simulink model "IEEE123bus_v2019b_Phasor_DPL"  (R2019b)
settings: Solver=VariableStepAuto  StartTime=0.0  StopTime=100  FixedStep=Ts  RelTol=1e-3
InitFcn:
  | a=1; % Loading Factor
  | Ts=0.1;% For Delay Blocks in Voltage Regulator Controls
  | 
  | % Simulation data for the IEEE 123 Node Test Feeder model
  | mi2km = 1.60934;%  miles to km conversion
  | ft2km = 0.0003048; % feet to km conversion
  | ms2F = 1*1e-6/(2*pi*60);% microsiemens to Farads conversion
  | 
  | %% Configuration 1
  | % Series Resitance and Reactance - ohm/mile
  | R_1 = [0.4576 0.1560 0.1535;0.1560 0.4666 0.1580;0.1535 0.1580 0.4615];
  | X_1 = [1.0780 0.5017 0.3849;0.5017 1.0482 0.4236;0.3849 0.4236 1.0651];
  | % charging susceptance - microsiemens/mile
  | B_1 = [5.6765 -1.8319 -0.6982;-1.8319 5.9809 -1.1645;-0.6982 -1.1645 5.3971];
  | 
  | R_1 = R_1/mi2km;
  | L_1 = (X_1/(2*pi*60))/mi2km;
  | C_1 =(B_1*ms2F)/mi2km;
  | 
  | %% Configuration 2 - series reactance - ohm/mile
  | R_2 = [0.4666 0.1580 0.1560;0.1580 0.4615 0.1535;0.1560 0.1535 0.4576];
  | X_2 = [1.0482 0.4236 0.5017;0.4236 1.0651 0.3849;0.5017 0.3849 1.0780];
  | % charging susceptance - microsiemens/mile
  | B_2 = [5.9809 -1.1645 -1.8319;-1.1645 5.3971 -0.6982;-1.8319 -0.6982 5.6765];
  | 
  | R_2 = R_2/mi2km;
  | L_2 = (X_2/(2*pi*60))/mi2km;
  | C_2 =(B_2*ms2F)/mi2km;
  | 
  | %% Configuration 3 - series reactance - ohm/mile
  | R_3 = [0.4615 0.1535 0.1580;0.1535 0.4576 0.1560;0.1580 0.1560 0.4666];
  | X_3 = [1.0651 0.3849 0.4236;0.3849 1.0780 0.5017;0.4236 0.5017 1.0482];
  | % charging susceptance - microsiemens/mile
  | B_3 = [5.3971 -0.6982 -1.1645;-0.6982 5.6765 -1.8319; -1.1645 -1.8319 5.9809];
  | 
  | R_3 = R_3/mi2km;
  | L_3 = (X_3/(2*pi*60))/mi2km;
  | C_3 =(B_3*ms2F)/mi2km;
  | 
  | %% Configuration 4 - series reactance - ohm/mile
  | R_4 = [0.4615 0.1580 0.1535;0.1580 0.4666 0.1560;0.1535 0.1560 0.4576];
  | X_4 = [1.0651 0.4236 0.3849;0.4236 1.0482 0.5017;0.3849 0.5017 1.0780];
  | % charging susceptance - microsiemens/mile
  | B_4 = [5.3971 -1.1645 -0.6982;-1.1645 5.9809 -1.8319;-0.6982 -1.8319 5.6765];
  | 
  | R_4 = R_4/mi2km;
  | L_4 = (X_4/(2*pi*60))/mi2km;
  | C_4 =(B_4*ms2F)/mi2km;
  | 
  | %% Configuration 5 - series reactance - ohm/mile
  | R_5 = [0.4666 0.1560 0.1580;0.1560 0.4576 0.1535;0.1580 0.1535 0.4615];
  | X_5 = [1.0482 0.5017 0.4236;0.5017 1.0780 0.3849;0.4236 0.3849 1.0651];
  | % charging susceptance - microsiemens/mile
  | B_5 = [5.9809 -1.8319 -1.1645;-1.8319 5.6765 -0.6982;-1.1645 -0.6982 5.3971];
  | 
  | R_5 = R_5/mi2km;
  | L_5 = (X_5/(2*pi*60))/mi2km;
  | C_5 =(B_5*ms2F)/mi2km;
  | 
  | %% Configuration 6 - series reactance - ohm/mile
  | R_6 = [0.4576 0.1535 0.1560;0.1535 0.4615 0.1580;0.1560 0.1580 0.4666];
  | X_6 = [1.0780 0.3849 0.5017;0.3849 1.0651 0.4236;0.5017 0.4236 1.0482];
  | % charging susceptance - microsiemens/mile
  | B_6 = [5.6765 -0.6982 -1.8319;-0.6982 5.3971 -1.1645;-1.8319 -1.1645 5.9809];
  | 
  | R_6 = R_6/mi2km;
  | L_6 = (X_6/(2*pi*60))/mi2km;
  | C_6 =(B_6*ms2F)/mi2km;
  | 
  | %% Configuration 7 - series reactance - ohm/mile
  | R_7 = [0.4576 0.0000 0.1535;0.0000 0.0000 0.0000;0.1535 0.0000 0.4615];
  | X_7 = [1.0780 0.0000 0.3849;0.0000 0.0000 0.0000;0.3849 0.0000 1.0651];
  | % charging susceptance - microsiemens/mile
  | B_7 = [5.1154 0.0000 -1.0549;0.0000 0.0000 0.0000;-1.0549 0.0000 5.1704];
  | 
  | R_7 = R_7/mi2km;
  | L_7 = (X_7/(2*pi*60))/mi2km;
  | C_7 =(B_7*ms2F)/mi2km;
  | 
  | %% Configuration 8 - series reactance - ohm/mile
  | R_8 = [0.4576 0.1535 0.0000;0.1535 0.4615 0.0000;0.0000 0.0000 0.0000];
  | X_8 = [1.0780 0.3849 0.0000;0.3849 1.0651 0.0000;0.0000 0.0000 0.0000];
  | % charging susceptance - microsiemens/mile
  | B_8 = [5.1154 -1.0549 0.0000;-1.0549 5.1704 0.0000;0.0000 0.0000 0.0000];
  | 
  | R_8 = R_8/mi2km;
  | L_8 = (X_8/(2*pi*60))/mi2km;
  | C_8 =(B_8*ms2F)/mi2km;
  | 
  | %% Configuration 9 - series reactance - ohm/mile
  | R_9 = [1.3292 0 0;0 0 0;0 0 0];
  | X_9 = [1.3475 0 0;0 0 0;0 0 0];
  | % charging susceptance - microsiemens/mile
  | B_9 = [4.5193 0 0;0 0 0;0 0 0];
  | 
  | R_9 = R_9/mi2km;
  | L_9 = (X_9/(2*pi*60))/mi2km;
  | C_9 =(B_9*ms2F)/mi2km;
  | 
  | %% Configuration 10- series reactance - ohm/mile
  | R_10 = [0 0 0;0 1.3292 0;0 0 0];
  | X_10 = [0 0 0;0 1.3475 0;0 0 0];
  | % charging susceptance - microsiemens/mile
  | B_10 = [0 0 0;0 4.5193 0;0 0 0];
  | 
  | R_10 = R_10/mi2km;
  | L_10 = (X_10/(2*pi*60))/mi2km;
  | C_10 =(B_10*ms2F)/mi2km;
  | 
  | %% Configuration 11 - series reactance - ohm/mile
  | R_11 = [0 0 0;0 0 0;0 0 1.3292];
  | X_11 = [0 0 0;0 0 0;0 0 1.3475];
  | % charging susceptance - microsiemens/mile
  | B_11 = [0 0 0;0 0 0;0 0 4.5193];
  | 
  | R_11 = R_11/mi2km;
  | L_11 = (X_11/(2*pi*60))/mi2km;
  | C_11 =(B_11*ms2F)/mi2km;
  | 
  | %% Configuration 12 - series reactance - ohm/mile
  | R_12 = [1.5209 0.5198 0.4924;0.5198 1.5329 0.5198;0.4924 0.5198 1.5209];
  | X_12 = [0.7521 0.2775 0.2157;0.2775 0.7162 0.2775;0.2157 0.2775 0.7521];
  | % charging susceptance - microsiemens/mile
  | B_12 = [67.2242 0.0000 0.0000;0.0000 67.2242 0.0000;0.0000 0.0000 67.2242];
  | 
  | R_12 = R_12/mi2km;
  | L_12 = (X_12/(2*pi*60))/mi2km;
  | C_12 =(B_12*ms2F)/mi2km;
undefined symbols (not defined in the file or in its folder): D1, Delta, find_system, j
libraries: powerlib x686, powerlib_meascontrol x31
(part 1 of 7)
settings Model: ARTEMISmethode_block_infos=$$__separator__$$pi123variableloadwith3PV/ARTEMIS Guide$$__separator__$$  Creator=Arun  LastModifiedBy=USARSUR
settings DataIOCC: ReturnWorkspaceOutputs=off
settings DebuggingCC: UnconnectedInputMsg=none  UnconnectedOutputMsg=none  UnconnectedLineMsg=none  ArithmeticOperatorsInVariantConditions=warning
settings SFSimCC: SimUseLocalCustomCode=off  CustomCodeUndefinedFunction=UseInterfaceOnly
settings RTWCC: RTWUseLocalCustomCode=off
settings CodeAppCC: StateflowObjectComments=on
settings SimscapeCC: SimscapeNormalizeSystem=off

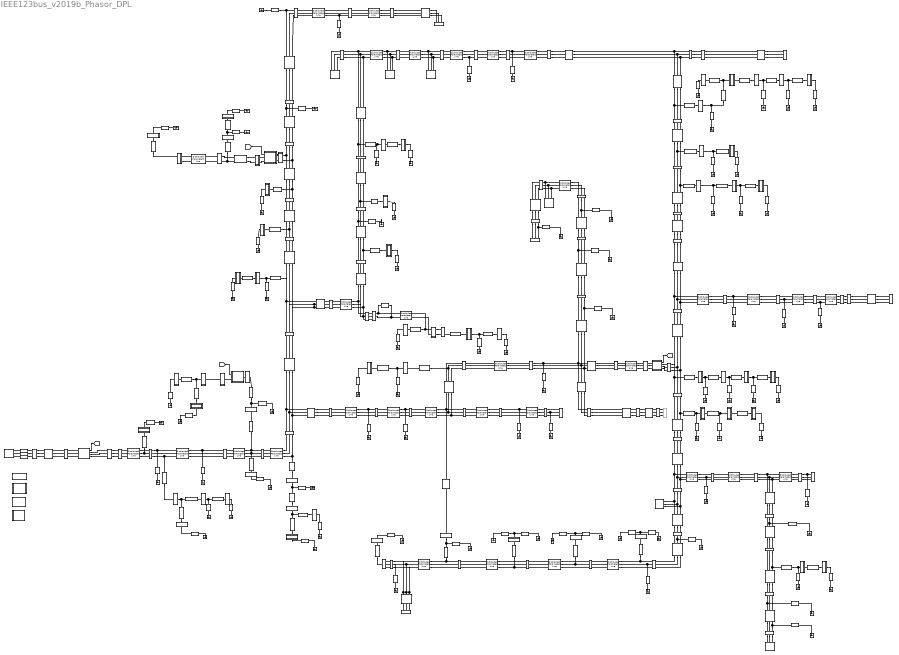
== system IEEE123bus_v2019b_Phasor_DPL ==
  note: Please consider citing following papers if the model was useful for your research
      |
      | A. Suresh, R. Bisht and S. Kamalasadan, "A Coordinated Control Architecture With Inverter-Based Resources and Legacy
      | Controllers of Power Distribution System for Voltage Profile Balance," in IEEE Transactions on Industry Applications, vol. 58,
      | no. 5, pp. 6701-6712, Sept.-Oct. 2022, doi: 10.1109/TIA.2022.3183030.
      |
      | A. Suresh, R. Bisht and S. Kamalasadan, "ADMM Based LQR for Voltage Regulation Using Distributed Energy Resources,"
      | 2020 IEEE International Conference on Power Electronics, Drives and Energy Systems (PEDES), 2020, pp. 1-6,
      | doi: 10.1109/PEDES49360.2020.9379625.
  note: Model Created by
      | Arun Suresh, Dr. Sukumar Kamalasadan,
      | University of North Carolina, Charlotte
  1 : powerlib/Measurements/Three-Phase V-I Measurement  VoltageMeasurement=phase-to-ground  SetLabelV=on  LabelV=V1  Vpu=off  VpuLL=off  CurrentMeasurement=no  SetLabelI=on  LabelI=I800  Ipu=off  Pbase=100e6  Vbase=24900  OutputType=Complex  PhasorSimulation=on  PSBequivalent=0
      settings: SourceProductName=Simscape Electrical
  1 Y PQ : powerlib/Elements/Series RLC Load  LConnTagsString=a  RConnTagsString=__new0  NominalVoltage=1.0*2401.78  NominalFrequency=60  ActivePower=40e3*a  InductivePower=20e3*a  CapacitivePower=0  Setx0=off  InitialVoltage=0  SetiL0=off  InitialCurrent=0  Measurements=None  LoadType=constant PQ
      settings: SourceProductName=Simscape Electrical
  1-2 10 : powerlib/Elements/Distributed Parameters Line  Phases=1  Frequency=60  Resistance=R_10(2,2)  Inductance=L_10(2,2)  Capacitance=C_10(2,2)  Length=175*ft2km  x1=[3380.56541461318;376.991118430775;-2.09963214230387]  x2=[3379.78750747913;376.991118430775;-2.09971060156131]  x3=[8.05427248749283;376.991118430775;0.227346207910768]  x4=[18.8407875620116;376.991118430775;-2.41591493087722]  x5=2.16957196133287e-07  V1=[2.049e+04;377;-2.115]  V2=[2.048e+04;377;-2.115]  I1=[33.62;377;-2.106]  I2=[35.2;377;-2.126]  nHarmo=1  Measurements=None
      settings: SourceProductName=Simscape Electrical
  1-3 11 : powerlib/Elements/Distributed Parameters Line  Phases=1  Frequency=60  Resistance=R_11(3,3)  Inductance=L_11(3,3)  Capacitance=C_11(3,3)  Length=250*ft2km  x1=[3361.50737999427;376.991118430775;2.08819907599433]  x2=[3355.99570274487;376.991118430775;2.08764080595054]  x3=[59.5194469552761;376.991118430775;-1.56433681880081]  x4=[70.5082076019166;376.991118430775;1.66262028833774]  x5=3.09938851618982e-07  V1=[2.049e+04;377;-2.115]  V2=[2.048e+04;377;-2.115]  I1=[33.62;377;-2.106]  I2=[35.2;377;-2.126]  nHarmo=1  Measurements=None
      settings: SourceProductName=Simscape Electrical
  1-7 1 : powerlib/Elements/Distributed Parameters Line  Phases=3  Frequency=60  Resistance=R_1  Inductance=L_1  Capacitance=C_1  Length=300*ft2km  x1=[418.369379874653 4119.59472126334 4115.60124511401;376.991118430775 376.991118430775 376.991118430775;1.71644980792441 -2.40630365835405 2.30078484563816]  x2=[407.597893112689 4096.26742166794 4094.04240143975;376.991118430775 376.991118430775 376.991118430775;1.73955161673438 -2.41014446431971 2.29348797562817]  x3=[123.925310729622 768.405747771136 838.862973764322;376.991118430775 376.991118430775 376.991118430775;2.95122481621433 0.252448117024993 -1.05952038647415]  x4=[123.559999451766 795.721759153579 862.519058134177;376.991118430775 376.991118430775 376.991118430775;-0.182106883383004 -2.87131680733943 2.08805814509585]  x5=3.76244991844366e-07  V1=ones(3,3)  V2=ones(3,3)  I1=ones(3,3)  I2=ones(3,3)  nHarmo=1  Measurements=None
      settings: SourceProductName=Simscape Electrical
  10 : Subsystem
  10 Y I : powerlib/Elements/Series RLC Load  LConnTagsString=a  RConnTagsString=__new0  NominalVoltage=1.0*2401.78  NominalFrequency=60  ActivePower=20e3*a  InductivePower=10e3*a  CapacitivePower=0  Setx0=off  InitialVoltage=0  SetiL0=off  InitialCurrent=0  Measurements=None  LoadType=constant I
      settings: SourceProductName=Simscape Electrical
  100 : powerlib/Measurements/Three-Phase V-I Measurement  VoltageMeasurement=phase-to-ground  SetLabelV=on  LabelV=V100  Vpu=off  VpuLL=off  CurrentMeasurement=no  SetLabelI=on  LabelI=I65  Ipu=off  Pbase=100e6  Vbase=24900  OutputType=Complex  PhasorSimulation=on  PSBequivalent=0
      settings: SourceProductName=Simscape Electrical
  100 Y Z : powerlib/Elements/Series RLC Load  LConnTagsString=a  RConnTagsString=__new0  NominalVoltage=1.0*2401.78  NominalFrequency=60  ActivePower=40e3*a  InductivePower=20e3*a  CapacitivePower=0  Setx0=off  InitialVoltage=0  SetiL0=off  InitialCurrent=0  Measurements=None  LoadType=constant Z
      settings: SourceProductName=Simscape Electrical
  100-450 3 : powerlib/Elements/Distributed Parameters Line  Phases=3  Frequency=60  Resistance=R_3  Inductance=L_3  Capacitance=C_3  Length=800*ft2km  x1=[406.131749441997 3939.12031039649 4017.5206124443;376.991118430775 376.991118430775 376.991118430775;-0.637933141409398 0.171201528668262 1.73700521240345]  x2=[406.131778494139 3939.12050268383 4017.52081027597;376.991118430775 376.991118430775 376.991118430775;-0.637933170107235 0.171201507341509 1.73700518522562]  x3=[0.533763849649707 11.60984734928 14.9950488986919;376.991118430775 376.991118430775 376.991118430775;-0.638311398489514 0.170889060671563 1.73669137648016]  x4=[0.533763849639262 11.6098473492939 14.9950488987535;376.991118430775 376.991118430775 376.991118430775;-0.637933170089052 0.171201507340757 1.73700518522527]  x5=1.00331997825164e-06  V1=ones(3,3)  V2=ones(3,3)  I1=ones(3,3)  I2=ones(3,3)  nHarmo=1  Measurements=None
      settings: SourceProductName=Simscape Electrical
  101 : powerlib/Measurements/Three-Phase V-I Measurement  VoltageMeasurement=phase-to-ground  SetLabelV=on  LabelV=V101  Vpu=off  VpuLL=off  CurrentMeasurement=no  SetLabelI=on  LabelI=I65  Ipu=off  Pbase=100e6  Vbase=24900  OutputType=Complex  PhasorSimulation=on  PSBequivalent=0
      settings: SourceProductName=Simscape Electrical
  101-102 11 : powerlib/Elements/Distributed Parameters Line  Phases=1  Frequency=60  Resistance=R_11(3,3)  Inductance=L_11(3,3)  Capacitance=C_11(3,3)  Length=225*ft2km  x1=[3251.35849286821;376.991118430775;2.0524184497167]  x2=[3246.56346361664;376.991118430775;2.05191677401351]  x3=[57.5262989800154;376.991118430775;-1.60039970533835]  x4=[68.1545739922667;376.991118430775;1.62666785892524]  x5=2.78944966457084e-07  V1=[2.049e+04;377;-2.115]  V2=[2.048e+04;377;-2.115]  I1=[33.62;377;-2.106]  I2=[35.2;377;-2.126]  nHarmo=1  Measurements=None
      settings: SourceProductName=Simscape Electrical
  101-105 3 : powerlib/Elements/Distributed Parameters Line  Phases=3  Frequency=60  Resistance=R_3  Inductance=L_3  Capacitance=C_3  Length=275*ft2km  x1=[403.657094793231 3937.42755462039 4018.23187990053;376.991118430775 376.991118430775 376.991118430775;-0.650924692497019 0.171464273667595 1.73744251449841]  x2=[403.635418531243 3934.47089431162 4016.39907349208;376.991118430775 376.991118430775 376.991118430775;-0.655781561403268 0.170968215664939 1.73704867653885]  x3=[17.9003688107967 79.6160512452646 59.5124978469701;376.991118430775 376.991118430775 376.991118430775;2.86937115405689 2.65811987542283 -1.846283722212]  x4=[18.8894010898735 99.0347590423608 87.5672430146078;376.991118430775 376.991118430775 376.991118430775;-0.293121067652145 -0.340334133509769 1.44230191886661]  x5=3.44891242524002e-07  V1=ones(3,3)  V2=ones(3,3)  I1=ones(3,3)  I2=ones(3,3)  nHarmo=1  Measurements=None
      settings: SourceProductName=Simscape Electrical
  102 : Subsystem
  102 Y Z : powerlib/Elements/Series RLC Load  LConnTagsString=a  RConnTagsString=__new0  NominalVoltage=1.0*2401.78  NominalFrequency=60  ActivePower=20e3*a  InductivePower=10e3*a  CapacitivePower=0  Setx0=off  InitialVoltage=0  SetiL0=off  InitialCurrent=0  Measurements=None  LoadType=constant Z
      settings: SourceProductName=Simscape Electrical
  102-103 11 : powerlib/Elements/Distributed Parameters Line  Phases=1  Frequency=60  Resistance=R_11(3,3)  Inductance=L_11(3,3)  Capacitance=C_11(3,3)  Length=325*ft2km  x1=[3246.56346361664;376.991118430775;2.05187003633578]  x2=[3241.0261246808;376.991118430775;2.05128908924918]  x3=[44.9655499069155;376.991118430775;-1.61347437800645]  x4=[55.5730572774;376.991118430775;1.63516683558841]  x5=4.02920507104677e-07  V1=[2.049e+04;377;-2.115]  V2=[2.048e+04;377;-2.115]  I1=[33.62;377;-2.106]  I2=[35.2;377;-2.126]  nHarmo=1  Measurements=None
      settings: SourceProductName=Simscape Electrical
  103 : Subsystem
  103 Y PQ : powerlib/Elements/Series RLC Load  LConnTagsString=a  RConnTagsString=__new0  NominalVoltage=1.0*2401.78  NominalFrequency=60  ActivePower=40e3*a  InductivePower=20e3*a  CapacitivePower=0  Setx0=off  InitialVoltage=0  SetiL0=off  InitialCurrent=0  Measurements=None  LoadType=constant PQ
      settings: SourceProductName=Simscape Electrical
  103-104 11 : powerlib/Elements/Distributed Parameters Line  Phases=1  Frequency=60  Resistance=R_11(3,3)  Inductance=L_11(3,3)  Capacitance=C_11(3,3)  Length=700*ft2km  x1=[3241.0261246808;376.991118430775;2.05111382295771]  x2=[3235.06887030603;376.991118430775;2.05048713201662]  x3=[19.9470002767371;376.991118430775;-1.68827039446278]  x4=[30.4892896750951;376.991118430775;1.67382868946066]  x5=8.6782878453315e-07  V1=[2.049e+04;377;-2.115]  V2=[2.048e+04;377;-2.115]  I1=[33.62;377;-2.106]  I2=[35.2;377;-2.126]  nHarmo=1  Measurements=None
      settings: SourceProductName=Simscape Electrical
  104 : Subsystem
  104 Y PQ : powerlib/Elements/Series RLC Load  LConnTagsString=a  RConnTagsString=__new0  NominalVoltage=1.0*2401.78  NominalFrequency=60  ActivePower=40e3*a  InductivePower=20e3*a  CapacitivePower=0  Setx0=off  InitialVoltage=0  SetiL0=off  InitialCurrent=0  Measurements=None  LoadType=constant PQ
      settings: SourceProductName=Simscape Electrical
  105 : powerlib/Measurements/Three-Phase V-I Measurement  VoltageMeasurement=phase-to-ground  SetLabelV=on  LabelV=V105  Vpu=off  VpuLL=off  CurrentMeasurement=no  SetLabelI=on  LabelI=I65  Ipu=off  Pbase=100e6  Vbase=24900  OutputType=Complex  PhasorSimulation=on  PSBequivalent=0
      settings: SourceProductName=Simscape Electrical
  105-106 10 : powerlib/Elements/Distributed Parameters Line  Phases=1  Frequency=60  Resistance=R_10(2,2)  Inductance=L_10(2,2)  Capacitance=C_10(2,2)  Length=225*ft2km  x1=[3304.98190011473;376.991118430775;-2.13405919078126]  x2=[3301.07685262134;376.991118430775;-2.13446171946558]  x3=[45.8104144500859;376.991118430775;0.484075429353889]  x4=[56.6127579803776;376.991118430775;-2.55054593205608]  x5=2.78944966457084e-07  V1=[2.049e+04;377;-2.115]  V2=[2.048e+04;377;-2.115]  I1=[33.62;377;-2.106]  I2=[35.2;377;-2.126]  nHarmo=1  Measurements=None
      settings: SourceProductName=Simscape Electrical
  105-108 3 : powerlib/Elements/Distributed Parameters Line  Phases=3  Frequency=60  Resistance=R_3  Inductance=L_3  Capacitance=C_3  Length=325*ft2km  x1=[403.635418531243 3934.47089431162 4016.39907349208;376.991118430775 376.991118430775 376.991118430775;-0.655805201573315 0.1709486870816 1.7370290626429]  x2=[402.074723888673 3931.7722646479 4016.56807334287;376.991118430775 376.991118430775 376.991118430775;-0.671182237047441 0.170609231399958 1.73692119301889]  x3=[50.1878882304407 55.6962408839422 11.7513473466765;376.991118430775 376.991118430775 376.991118430775;2.61416246353745 2.47843227593797 0.843207511127157]  x4=[51.2372486550466 73.3161862808586 24.4058651044384;376.991118430775 376.991118430775 376.991118430775;-0.530234910581878 -0.426773816811748 2.12160754968628]  x5=4.0759874116473e-07  V1=ones(3,3)  V2=ones(3,3)  I1=ones(3,3)  I2=ones(3,3)  nHarmo=1  Measurements=None
      settings: SourceProductName=Simscape Electrical
  106 : Subsystem
  106 Y PQ : powerlib/Elements/Series RLC Load  LConnTagsString=a  RConnTagsString=__new0  NominalVoltage=1.0*2401.78  NominalFrequency=60  ActivePower=40e3*a  InductivePower=20e3*a  CapacitivePower=0  Setx0=off  InitialVoltage=0  SetiL0=off  InitialCurrent=0  Measurements=None  LoadType=constant PQ
      settings: SourceProductName=Simscape Electrical
  106-107 10 : powerlib/Elements/Distributed Parameters Line  Phases=1  Frequency=60  Resistance=R_10(2,2)  Inductance=L_10(2,2)  Capacitance=C_10(2,2)  Length=575*ft2km  x1=[3301.07685262134;376.991118430775;-2.13462530133762]  x2=[3296.09115865668;376.991118430775;-2.13514024446439]  x3=[20.3252283129498;376.991118430775;0.40935318589622]  x4=[31.0653774222284;376.991118430775;-2.51179765756046]  x5=7.12859358723659e-07  V1=[2.049e+04;377;-2.115]  V2=[2.048e+04;377;-2.115]  I1=[33.62;377;-2.106]  I2=[35.2;377;-2.126]  nHarmo=1  Measurements=None
      settings: SourceProductName=Simscape Electrical
  107 : Subsystem
  107 Y PQ : powerlib/Elements/Series RLC Load  LConnTagsString=a  RConnTagsString=__new0  NominalVoltage=1.0*2401.78  NominalFrequency=60  ActivePower=40e3*a  InductivePower=20e3*a  CapacitivePower=0  Setx0=off  InitialVoltage=0  SetiL0=off  InitialCurrent=0  Measurements=None  LoadType=constant PQ
      settings: SourceProductName=Simscape Electrical
  108 : powerlib/Measurements/Three-Phase V-I Measurement  VoltageMeasurement=phase-to-ground  SetLabelV=on  LabelV=V108  Vpu=off  VpuLL=off  CurrentMeasurement=no  SetLabelI=on  LabelI=I65  Ipu=off  Pbase=100e6  Vbase=24900  OutputType=Complex  PhasorSimulation=on  PSBequivalent=0
      settings: SourceProductName=Simscape Electrical
  108-109 9 : powerlib/Elements/Distributed Parameters Line  Phases=1  Frequency=60  Resistance=R_9(1,1)  Inductance=L_9(1,1)  Capacitance=C_9(1,1)  Length=450*ft2km  x1=[3181.15673359339;376.991118430775;-0.0628869901083998]  x2=[3168.06194978621;376.991118430775;-0.0642859616608475]  x3=[80.5463139182893;376.991118430775;2.58026488742804]  x4=[90.9315802089911;376.991118430775;-0.500259322316593]  x5=5.57889932914168e-07  V1=[2.049e+04;377;-2.115]  V2=[2.048e+04;377;-2.115]  I1=[33.62;377;-2.106]  I2=[35.2;377;-2.126]  nHarmo=1  Measurements=None
      settings: SourceProductName=Simscape Electrical
  108-300 3 : powerlib/Elements/Distributed Parameters Line  Phases=3  Frequency=60  Resistance=R_3  Inductance=L_3  Capacitance=C_3  Length=1000*ft2km  x1=[402.074723888673 3931.7722646479 4016.56807334287;376.991118430775 376.991118430775 376.991118430775;-0.671501379343069 0.170345595524886 1.73665640542353]  x2=[402.074761358754 3931.77255721669 4016.56837602683;376.991118430775 376.991118430775 376.991118430775;-0.671501420907049 0.170345564472289 1.73665636432255]  x3=[0.528412808323245 11.5879303032605 14.9910215576854;376.991118430775 376.991118430775 376.991118430775;-0.671937963049553 0.169961143904011 1.73626866977983]  x4=[0.528420850969568 11.5878577029287 14.9909927851014;376.991118430775 376.991118430775 376.991118430775;-0.671537666068559 0.170339428949189 1.73665180118272]  x5=1.25414997281455e-06  V1=ones(3,3)  V2=ones(3,3)  I1=ones(3,3)  I2=ones(3,3)  nHarmo=1  Measurements=None
      settings: SourceProductName=Simscape Electrical
  109 : Subsystem
  109 Y PQ : powerlib/Elements/Series RLC Load  LConnTagsString=a  RConnTagsString=__new0  NominalVoltage=1.0*2401.78  NominalFrequency=60  ActivePower=40e3*a  InductivePower=20e3*a  CapacitivePower=0  Setx0=off  InitialVoltage=0  SetiL0=off  InitialCurrent=0  Measurements=None  LoadType=constant PQ
      settings: SourceProductName=Simscape Electrical
  109-110 9 : powerlib/Elements/Distributed Parameters Line  Phases=1  Frequency=60  Resistance=R_9(1,1)  Inductance=L_9(1,1)  Capacitance=C_9(1,1)  Length=300*ft2km  x1=[3168.06194978621;376.991118430775;-0.0642158551442573]  x2=[3161.83483122911;376.991118430775;-0.064884594025442]  x3=[56.0271358889941;376.991118430775;2.56601096641357]  x4=[66.3801617084479;376.991118430775;-0.490087419533799]  x5=3.71926621942778e-07  V1=[2.049e+04;377;-2.115]  V2=[2.048e+04;377;-2.115]  I1=[33.62;377;-2.106]  I2=[35.2;377;-2.126]  nHarmo=1  Measurements=None
      settings: SourceProductName=Simscape Electrical
  11 : Subsystem
  11 Y Z : powerlib/Elements/Series RLC Load  LConnTagsString=a  RConnTagsString=__new0  NominalVoltage=1.0*2401.78  NominalFrequency=60  ActivePower=40e3*a  InductivePower=20e3*a  CapacitivePower=0  Setx0=off  InitialVoltage=0  SetiL0=off  InitialCurrent=0  Measurements=None  LoadType=constant Z
      settings: SourceProductName=Simscape Electrical
  110 : Subsystem
  110-111 9 : powerlib/Elements/Distributed Parameters Line  Phases=1  Frequency=60  Resistance=R_9(1,1)  Inductance=L_9(1,1)  Capacitance=C_9(1,1)  Length=575*ft2km  x1=[3161.83483122911;376.991118430775;-0.0650131226391907]  x2=[3159.44549174791;376.991118430775;-0.0652708065834279]  x3=[7.52655039714254;376.991118430775;2.26152167646501]  x4=[17.6106029911177;376.991118430775;-0.381479851658474]  x5=7.12859358723659e-07  V1=[2.049e+04;377;-2.115]  V2=[2.048e+04;377;-2.115]  I1=[33.62;377;-2.106]  I2=[35.2;377;-2.126]  nHarmo=1  Measurements=None
      settings: SourceProductName=Simscape Electrical
  110-112 9 : powerlib/Elements/Distributed Parameters Line  Phases=1  Frequency=60  Resistance=R_9(1,1)  Inductance=L_9(1,1)  Capacitance=C_9(1,1)  Length=125*ft2km  x1=[3161.83483122911;376.991118430775;-0.0648028030894201]  x2=[3159.75997373429;376.991118430775;-0.0650261502258887]  x3=[43.8089246818886;376.991118430775;2.55317269137536]  x4=[54.1453656807879;376.991118430775;-0.481335615539711]  x5=1.54969425809491e-07  V1=[2.049e+04;377;-2.115]  V2=[2.048e+04;377;-2.115]  I1=[33.62;377;-2.106]  I2=[35.2;377;-2.126]  nHarmo=1  Measurements=None
      settings: SourceProductName=Simscape Electrical
  111 : Subsystem
  111 Y PQ : powerlib/Elements/Series RLC Load  LConnTagsString=a  RConnTagsString=__new0  NominalVoltage=1.0*2401.78  NominalFrequency=60  ActivePower=20e3*a  InductivePower=10e3*a  CapacitivePower=0  Setx0=off  InitialVoltage=0  SetiL0=off  InitialCurrent=0  Measurements=None  LoadType=constant PQ
      settings: SourceProductName=Simscape Electrical
  112 : Subsystem
  112 Y I : powerlib/Elements/Series RLC Load  LConnTagsString=a  RConnTagsString=__new0  NominalVoltage=1.0*2401.78  NominalFrequency=60  ActivePower=20e3*a  InductivePower=10e3*a  CapacitivePower=0  Setx0=off  InitialVoltage=0  SetiL0=off  InitialCurrent=0  Measurements=None  LoadType=constant I
      settings: SourceProductName=Simscape Electrical
  112-113 9 : powerlib/Elements/Distributed Parameters Line  Phases=1  Frequency=60  Resistance=R_9(1,1)  Inductance=L_9(1,1)  Capacitance=C_9(1,1)  Length=525*ft2km  x1=[3159.75997373429;376.991118430775;-0.0652131009367958]  x2=[3153.22836502941;376.991118430775;-0.0659177727875796]  x3=[31.5914511772632;376.991118430775;2.52992679657941]  x4=[41.9022702912703;376.991118430775;-0.467929617642989]  x5=6.50871588399862e-07  V1=[2.049e+04;377;-2.115]  V2=[2.048e+04;377;-2.115]  I1=[33.62;377;-2.106]  I2=[35.2;377;-2.126]  nHarmo=1  Measurements=None
      settings: SourceProductName=Simscape Electrical
  113 : Subsystem
  113 Y Z : powerlib/Elements/Series RLC Load  LConnTagsString=a  RConnTagsString=__new0  NominalVoltage=1.0*2401.78  NominalFrequency=60  ActivePower=40e3*a  InductivePower=20e3*a  CapacitivePower=0  Setx0=off  InitialVoltage=0  SetiL0=off  InitialCurrent=0  Measurements=None  LoadType=constant PQ
      settings: SourceProductName=Simscape Electrical
  113-114 9 : powerlib/Elements/Distributed Parameters Line  Phases=1  Frequency=60  Resistance=R_9(1,1)  Inductance=L_9(1,1)  Capacitance=C_9(1,1)  Length=325*ft2km  x1=[3153.22836502941;376.991118430775;-0.065824297432126]  x2=[3151.88109992036;376.991118430775;-0.065969983994272]  x3=[7.51017087819426;376.991118430775;2.26098770058323]  x4=[17.569609951979;376.991118430775;-0.382176085871868]  x5=4.02920507104677e-07  V1=[2.049e+04;377;-2.115]  V2=[2.048e+04;377;-2.115]  I1=[33.62;377;-2.106]  I2=[35.2;377;-2.126]  nHarmo=1  Measurements=None
      settings: SourceProductName=Simscape Electrical
  114 : Subsystem
  114 Y PQ : powerlib/Elements/Series RLC Load  LConnTagsString=a  RConnTagsString=__new0  NominalVoltage=1.0*2401.78  NominalFrequency=60  ActivePower=20e3*a  InductivePower=10e3*a  CapacitivePower=0  Setx0=off  InitialVoltage=0  SetiL0=off  InitialCurrent=0  Measurements=None  LoadType=constant PQ
      settings: SourceProductName=Simscape Electrical
  12 : Subsystem
  12 Y PQ : powerlib/Elements/Series RLC Load  LConnTagsString=a  RConnTagsString=__new0  NominalVoltage=1.0*2401.78  NominalFrequency=60  ActivePower=20e3*a  InductivePower=10e3*a  CapacitivePower=0  Setx0=off  InitialVoltage=0  SetiL0=off  InitialCurrent=0  Measurements=None  LoadType=constant PQ
      settings: SourceProductName=Simscape Electrical
  13 : powerlib/Measurements/Three-Phase V-I Measurement  VoltageMeasurement=phase-to-ground  SetLabelV=on  LabelV=V13  Vpu=off  VpuLL=off  CurrentMeasurement=no  SetLabelI=on  LabelI=I800  Ipu=off  Pbase=100e6  Vbase=24900  OutputType=Complex  PhasorSimulation=on  PSBequivalent=0
      settings: SourceProductName=Simscape Electrical
  13-152 : powerlib/Elements/Three-Phase Breaker  InitialState=closed  SwitchA=off  SwitchB=off  SwitchC=off  SwitchTimes=50  External=off  BreakerResistance=0.01  SnubberResistance=1e6  SnubberCapacitance=inf  Measurements=None
      settings: SourceProductName=Simscape Electrical
  13-18 2 : powerlib/Elements/Distributed Parameters Line  Phases=3  Frequency=60  Resistance=R_2  Inductance=L_2  Capacitance=C_2  Length=825*ft2km  x1=[478.852724771023 4035.93644364242 4080.83240152102;376.991118430775 376.991118430775 376.991118430775;-2.48395100094719 -0.333291624454928 -1.89649172656706]  x2=[492.987972620977 4009.26229356499 4052.37399314383;376.991118430775 376.991118430775 376.991118430775;-2.48166557625713 -0.338166239287337 -1.90023995127769]  x3=[44.6237708036965 320.691471267729 261.273246184064;376.991118430775 376.991118430775 376.991118430775;2.70213633371866 2.35350354720008 0.547506552689311]  x4=[44.0568895422193 347.948500447661 280.097141126017;376.991118430775 376.991118430775 376.991118430775;-0.465270555224082 -0.750371469449044 -2.53921646273606]  x5=1.03467372757201e-06  V1=ones(3,3)  V2=ones(3,3)  I1=ones(3,3)  I2=ones(3,3)  nHarmo=1  Measurements=None
      settings: SourceProductName=Simscape Electrical
  13-34 11 : powerlib/Elements/Distributed Parameters Line  Phases=1  Frequency=60  Resistance=R_11(3,3)  Inductance=L_11(3,3)  Capacitance=C_11(3,3)  Length=150*ft2km  x1=[3314.02445205709;376.991118430775;2.07559914731532]  x2=[3310.76065547735;376.991118430775;2.07526361506547]  x3=[58.7539638219961;376.991118430775;-1.57644134792345]  x4=[69.5930366178704;376.991118430775;1.65039230220132]  x5=1.85963310971389e-07  V1=[2.049e+04;377;-2.115]  V2=[2.048e+04;377;-2.115]  I1=[33.62;377;-2.106]  I2=[35.2;377;-2.126]  nHarmo=1  Measurements=None
      settings: SourceProductName=Simscape Electrical
  135 : powerlib/Measurements/Three-Phase V-I Measurement  VoltageMeasurement=phase-to-ground  SetLabelV=on  LabelV=V135  Vpu=off  VpuLL=off  CurrentMeasurement=no  SetLabelI=on  LabelI=I800  Ipu=off  Pbase=100e6  Vbase=24900  OutputType=Complex  PhasorSimulation=on  PSBequivalent=0
      settings: SourceProductName=Simscape Electrical
  135-35 4 : powerlib/Elements/Distributed Parameters Line  Phases=3  Frequency=60  Resistance=R_4  Inductance=L_4  Capacitance=C_4  Length=375*ft2km  x1=[358.201071745182 4002.76233206844 4057.33772493146;376.991118430775 376.991118430775 376.991118430775;0.288428319237875 -0.244778865053432 -1.80945312237022]  x2=[355.896463859393 3994.45012863587 4048.64412017082;376.991118430775 376.991118430775 376.991118430775;0.294347808818621 -0.246670597461798 -1.81030589171295]  x3=[21.6836637125812 196.552740350504 196.379296794755;376.991118430775 376.991118430775 376.991118430775;1.48118471514768 2.45073860387519 0.594623029419391]  x4=[21.3525295771726 218.064396683571 219.726877596892;376.991118430775 376.991118430775 376.991118430775;-1.61959125907542 -0.644301438757731 -2.45428955376116]  x5=4.70306239805458e-07  V1=ones(3,3)  V2=ones(3,3)  I1=ones(3,3)  I2=ones(3,3)  nHarmo=1  Measurements=None
      settings: SourceProductName=Simscape Electrical
  14 : Subsystem
  14-10 9 : powerlib/Elements/Distributed Parameters Line  Phases=1  Frequency=60  Resistance=R_9(1,1)  Inductance=L_9(1,1)  Capacitance=C_9(1,1)  Length=250*ft2km  x1=[3286.69613198261;376.991118430775;-0.0232422684147907]  x2=[3287.77681830584;376.991118430775;-0.0231301927977185]  x3=[18.3214789637549;376.991118430775;-0.339447487298582]  x4=[7.83191582671298;376.991118430775;2.30376497126479]  x5=3.09938851618982e-07  V1=[2.049e+04;377;-2.115]  V2=[2.048e+04;377;-2.115]  I1=[33.62;377;-2.106]  I2=[35.2;377;-2.126]  nHarmo=1  Measurements=None
      settings: SourceProductName=Simscape Electrical
  14-11 9 : powerlib/Elements/Distributed Parameters Line  Phases=1  Frequency=60  Resistance=R_9(1,1)  Inductance=L_9(1,1)  Capacitance=C_9(1,1)  Length=250*ft2km  x1=[3287.77681830584;376.991118430775;-0.0231301927977185]  x2=[3285.61609222663;376.991118430775;-0.0233542636458793]  x3=[20.2657478497464;376.991118430775;2.52130984001914]  x4=[30.9691803951139;376.991118430775;-0.400009000192558]  x5=3.09938851618982e-07  V1=[2.049e+04;377;-2.115]  V2=[2.048e+04;377;-2.115]  I1=[33.62;377;-2.106]  I2=[35.2;377;-2.126]  nHarmo=1  Measurements=None
      settings: SourceProductName=Simscape Electrical
  149 : powerlib/Measurements/Three-Phase V-I Measurement  VoltageMeasurement=phase-to-ground  SetLabelV=on  LabelV=V149  Vpu=off  VpuLL=off  CurrentMeasurement=no  SetLabelI=on  LabelI=I800  Ipu=off  Pbase=100e6  Vbase=24900  OutputType=Complex  PhasorSimulation=on  PSBequivalent=0
      settings: SourceProductName=Simscape Electrical
  149-1 1 : powerlib/Elements/Distributed Parameters Line  Phases=3  Frequency=60  Resistance=R_1  Inductance=L_1  Capacitance=C_1  Length=400*ft2km  x1=[435.805362277063 4151.64661830078 4147.4219015932;376.991118430775 376.991118430775 376.991118430775;1.69509188651091 -2.40112016359797 2.31085182357606]  x2=[418.369379874653 4119.59472126334 4115.60124511402;376.991118430775 376.991118430775 376.991118430775;1.71640252758432 -2.40634288614596 2.30074578847149]  x3=[126.910577019072 791.236572596697 895.735122488467;376.991118430775 376.991118430775 376.991118430775;-3.11071954514432 0.255388857840873 -1.07839958942856]  x4=[126.799213786087 818.712230576718 919.395559444508;376.991118430775 376.991118430775 376.991118430775;0.0396790486071372 -2.86870887855285 2.06955534618551]  x5=5.01659989125821e-07  V1=ones(3,3)  V2=ones(3,3)  I1=ones(3,3)  I2=ones(3,3)  nHarmo=1  Measurements=None
      settings: SourceProductName=Simscape Electrical
  15 : Subsystem
  15-16 11 : powerlib/Elements/Distributed Parameters Line  Phases=1  Frequency=60  Resistance=R_11(3,3)  Inductance=L_11(3,3)  Capacitance=C_11(3,3)  Length=375*ft2km  x1=[3309.45581098444;376.991118430775;2.07502418259757]  x2=[3306.19437716597;376.991118430775;2.07468818168711]  x3=[20.3906959030593;376.991118430775;-1.6638986627683]  x4=[31.1621657776187;376.991118430775;1.6980324157015]  x5=4.64908277428473e-07  V1=[2.049e+04;377;-2.115]  V2=[2.048e+04;377;-2.115]  I1=[33.62;377;-2.106]  I2=[35.2;377;-2.126]  nHarmo=1  Measurements=None
      settings: SourceProductName=Simscape Electrical
  15-17 11 : powerlib/Elements/Distributed Parameters Line  Phases=1  Frequency=60  Resistance=R_11(3,3)  Inductance=L_11(3,3)  Capacitance=C_11(3,3)  Length=350*ft2km  x1=[3309.45581098444;376.991118430775;2.075035867017]  x2=[3307.93307517121;376.991118430775;2.07487897801]  x3=[7.88183281420355;376.991118430775;-1.88136516351838]  x4=[18.4393715425204;376.991118430775;1.75867258184176]  x5=4.33914392266575e-07  V1=[2.049e+04;377;-2.115]  V2=[2.048e+04;377;-2.115]  I1=[33.62;377;-2.106]  I2=[35.2;377;-2.126]  nHarmo=1  Measurements=None
      settings: SourceProductName=Simscape Electrical
  150 : powerlib/Measurements/Three-Phase V-I Measurement  VoltageMeasurement=phase-to-ground  SetLabelV=on  LabelV=V150  Vpu=off  VpuLL=off  CurrentMeasurement=yes  SetLabelI=on  LabelI=I150  Ipu=off  Pbase=100e6  Vbase=24900  OutputType=Complex  PhasorSimulation=on  PSBequivalent=0
      settings: SourceProductName=Simscape Electrical
  150-1 : powerlib/Elements/Three-Phase Breaker  InitialState=closed  SwitchA=off  SwitchB=off  SwitchC=off  SwitchTimes="[1/60  5/60]"  External=off  BreakerResistance=0.01  SnubberResistance=1e6  SnubberCapacitance=inf  Measurements=None
      settings: SourceProductName=Simscape Electrical
  151 : powerlib/Measurements/Three-Phase V-I Measurement  VoltageMeasurement=phase-to-ground  SetLabelV=on  LabelV=V151  Vpu=off  VpuLL=off  CurrentMeasurement=no  SetLabelI=on  LabelI=I65  Ipu=off  Pbase=100e6  Vbase=24900  OutputType=Complex  PhasorSimulation=on  PSBequivalent=0
      settings: SourceProductName=Simscape Electrical
  151-1 : powerlib/Elements/Three-Phase Breaker  InitialState=open  SwitchA=off  SwitchB=off  SwitchC=off  SwitchTimes="[1/60  5/60]"  External=off  BreakerResistance=0.01  SnubberResistance=1e6  SnubberCapacitance=inf  Measurements=None
      settings: SourceProductName=Simscape Electrical
  152 : powerlib/Measurements/Three-Phase V-I Measurement  VoltageMeasurement=phase-to-ground  SetLabelV=on  LabelV=V152  Vpu=off  VpuLL=off  CurrentMeasurement=no  SetLabelI=on  LabelI=I65  Ipu=off  Pbase=100e6  Vbase=24900  OutputType=Complex  PhasorSimulation=on  PSBequivalent=0
      settings: SourceProductName=Simscape Electrical
  152-52 1 : powerlib/Elements/Distributed Parameters Line  Phases=3  Frequency=60  Resistance=R_1  Inductance=L_1  Capacitance=C_1  Length=400*ft2km  x1=[391.941447057197 4055.20520317865 4054.05664372454;376.991118430775 376.991118430775 376.991118430775;1.76902090571785 -2.41636953562623 2.28175286760386]  x2=[387.990472092363 4040.29436483784 4040.67700374777;376.991118430775 376.991118430775 376.991118430775;1.78456610468743 -2.42012059741259 2.27569658683885]  x3=[46.966631603242 428.664477419494 470.902529588853;376.991118430775 376.991118430775 376.991118430775;2.72688224247446 0.441773514605444 -0.952909754634023]  x4=[46.3780537809962 457.769746242821 494.66955794637;376.991118430775 376.991118430775 376.991118430775;-0.396728206021515 -2.6814806252105 2.19301642793857]  x5=5.01659989125821e-07  V1=ones(3,3)  V2=ones(3,3)  I1=ones(3,3)  I2=ones(3,3)  nHarmo=1  Measurements=None
      settings: SourceProductName=Simscape Electrical
  16 : Subsystem
  16 Y PQ : powerlib/Elements/Series RLC Load  LConnTagsString=a  RConnTagsString=__new0  NominalVoltage=1.0*2401.78  NominalFrequency=60  ActivePower=40e3*a  InductivePower=20e3*a  CapacitivePower=0  Setx0=off  InitialVoltage=0  SetiL0=off  InitialCurrent=0  Measurements=None  LoadType=constant PQ
      settings: SourceProductName=Simscape Electrical
  160 : powerlib/Measurements/Three-Phase V-I Measurement  VoltageMeasurement=phase-to-ground  SetLabelV=on  LabelV=V160  Vpu=off  VpuLL=off  CurrentMeasurement=no  SetLabelI=on  LabelI=I65  Ipu=off  Pbase=100e6  Vbase=24900  OutputType=Complex  PhasorSimulation=on  PSBequivalent=0
      settings: SourceProductName=Simscape Electrical
  160 67 6 : powerlib/Elements/Distributed Parameters Line  Phases=3  Frequency=60  Resistance=R_3  Inductance=L_3  Capacitance=C_3  Length=350*ft2km  x1=[404.538488613554 3952.714067319 4028.61066081034;376.991118430775 376.991118430775 376.991118430775;-0.628407351241529 0.176232710670968 1.74112907171472]  x2=[404.043073896034 3944.41296070391 4023.02737587841;376.991118430775 376.991118430775 376.991118430775;-0.642056014650593 0.1723902350794 1.73819837777504]  x3=[40.3301494195195 330.117850016404 295.684253134342;376.991118430775 376.991118430775 376.991118430775;2.80205327966435 -3.05920638037755 -1.33651203404679]  x4=[41.3478953990251 353.302821549694 325.679980992776;376.991118430775 376.991118430775 376.991118430775;-0.347031052737195 0.0884297417604716 1.79904189655825]  x5=4.38952490485094e-07  V1=ones(3,3)  V2=ones(3,3)  I1=ones(3,3)  I2=ones(3,3)  nHarmo=1  Measurements=None
      settings: SourceProductName=Simscape Electrical
  17 : Subsystem
  17 Y PQ : powerlib/Elements/Series RLC Load  LConnTagsString=a  RConnTagsString=__new0  NominalVoltage=1.0*2401.78  NominalFrequency=60  ActivePower=20e3*a  InductivePower=10e3*a  CapacitivePower=0  Setx0=off  InitialVoltage=0  SetiL0=off  InitialCurrent=0  Measurements=None  LoadType=constant PQ
      settings: SourceProductName=Simscape Electrical
  18 : powerlib/Measurements/Three-Phase V-I Measurement  VoltageMeasurement=phase-to-ground  SetLabelV=on  LabelV=V18  Vpu=off  VpuLL=off  CurrentMeasurement=no  SetLabelI=on  LabelI=I800  Ipu=off  Pbase=100e6  Vbase=24900  OutputType=Complex  PhasorSimulation=on  PSBequivalent=0
      settings: SourceProductName=Simscape Electrical
  18-135 : powerlib/Elements/Three-Phase Breaker  InitialState=closed  SwitchA=off  SwitchB=off  SwitchC=off  SwitchTimes=10  External=off  BreakerResistance=0.01  SnubberResistance=1e6  SnubberCapacitance=inf  Measurements=None
      settings: SourceProductName=Simscape Electrical
  18-19 9 : powerlib/Elements/Distributed Parameters Line  Phases=1  Frequency=60  Resistance=R_9(1,1)  Inductance=L_9(1,1)  Capacitance=C_9(1,1)  Length=250*ft2km  x1=[3243.01279991712;376.991118430775;-0.0362645602700382]  x2=[3238.75445154485;376.991118430775;-0.0367120365752278]  x3=[44.961322061258;376.991118430775;2.58194504165251]  x4=[55.5607503638828;376.991118430775;-0.45272188075142]  x5=3.09938851618982e-07  V1=[2.049e+04;377;-2.115]  V2=[2.048e+04;377;-2.115]  I1=[33.62;377;-2.106]  I2=[35.2;377;-2.126]  nHarmo=1  Measurements=None
      settings: SourceProductName=Simscape Electrical
  18-21 2 : powerlib/Elements/Distributed Parameters Line  Phases=3  Frequency=60  Resistance=R_2  Inductance=L_2  Capacitance=C_2  Length=300*ft2km  x1=[492.987972620977 4009.26229356499 4052.37399314383;376.991118430775 376.991118430775 376.991118430775;-2.48141735447164 -0.337960293379835 -1.90003490115264]  x2=[494.38975347698 4006.40018891149 4050.73705232197;376.991118430775 376.991118430775 376.991118430775;-2.4755487250542 -0.338371736117516 -1.90048804357191]  x3=[28.3270843908106 79.3019052360677 45.5017429231014;376.991118430775 376.991118430775 376.991118430775;-2.54607461055668 2.16182672364167 0.843292098242158]  x4=[27.0324232804458 104.813878446454 68.1506319927301;376.991118430775 376.991118430775 376.991118430775;0.592278799269531 -0.808095741348943 -2.16205651826691]  x5=3.76244991844366e-07  V1=ones(3,3)  V2=ones(3,3)  I1=ones(3,3)  I2=ones(3,3)  nHarmo=1  Measurements=None
      settings: SourceProductName=Simscape Electrical
  19 : Subsystem
  19 Y PQ : powerlib/Elements/Series RLC Load  LConnTagsString=a  RConnTagsString=__new0  NominalVoltage=1.0*2401.78  NominalFrequency=60  ActivePower=40e3*a  InductivePower=20e3*a  CapacitivePower=0  Setx0=off  InitialVoltage=0  SetiL0=off  InitialCurrent=0  Measurements=None  LoadType=constant PQ
      settings: SourceProductName=Simscape Electrical
  19-20 9 : powerlib/Elements/Distributed Parameters Line  Phases=1  Frequency=60  Resistance=R_9(1,1)  Inductance=L_9(1,1)  Capacitance=C_9(1,1)  Length=325*ft2km  x1=[3238.75445154485;376.991118430775;-0.0367470898335229]  x2=[3235.98791276244;376.991118430775;-0.037038327131086]  x3=[19.9584780005766;376.991118430775;2.50758637721562]  x4=[30.5008259417973;376.991118430775;-0.413693691919667]  x5=4.02920507104677e-07  V1=[2.049e+04;377;-2.115]  V2=[2.048e+04;377;-2.115]  I1=[33.62;377;-2.106]  I2=[35.2;377;-2.126]  nHarmo=1  Measurements=None
      settings: SourceProductName=Simscape Electrical
  197 : powerlib/Measurements/Three-Phase V-I Measurement  VoltageMeasurement=phase-to-ground  SetLabelV=on  LabelV=V197  Vpu=off  VpuLL=off  CurrentMeasurement=no  SetLabelI=on  LabelI=I65  Ipu=off  Pbase=100e6  Vbase=24900  OutputType=Complex  PhasorSimulation=on  PSBequivalent=0
      settings: SourceProductName=Simscape Electrical
  197-101 3 : powerlib/Elements/Distributed Parameters Line  Phases=3  Frequency=60  Resistance=R_3  Inductance=L_3  Capacitance=C_3  Length=250*ft2km  x1=[403.685053346447 3940.11622916439 4019.89856666797;376.991118430775 376.991118430775 376.991118430775;-0.646498059979194 0.171924358696273 1.73781004953439]  x2=[403.657094793231 3937.42755462039 4018.23187990053;376.991118430775 376.991118430775 376.991118430775;-0.650912872411995 0.171474037959265 1.73745232144639]  x3=[17.8996095188031 79.6124912221135 59.5086432134533;376.991118430775 376.991118430775 376.991118430775;2.86926713192411 2.65802869813203 -1.84637830521527]  x4=[18.8904762438731 99.0392285204412 87.5718139939841;376.991118430775 376.991118430775 376.991118430775;-0.292976913980804 -0.340219226209111 1.44241655086083]  x5=3.13537493203638e-07  V1=ones(3,3)  V2=ones(3,3)  I1=ones(3,3)  I2=ones(3,3)  nHarmo=1  Measurements=None
      settings: SourceProductName=Simscape Electrical
  2 : Subsystem
  2 Y PQ : powerlib/Elements/Series RLC Load  LConnTagsString=a  RConnTagsString=__new0  NominalVoltage=1.0*2401.78  NominalFrequency=60  ActivePower=20e3*a  InductivePower=10e3*a  CapacitivePower=0  Setx0=off  InitialVoltage=0  SetiL0=off  InitialCurrent=0  Measurements=None  LoadType=constant PQ
      settings: SourceProductName=Simscape Electrical
  20 : Subsystem
  20 Y I : powerlib/Elements/Series RLC Load  LConnTagsString=a  RConnTagsString=__new0  NominalVoltage=1.0*2401.78  NominalFrequency=60  ActivePower=40e3*a  InductivePower=20e3*a  CapacitivePower=0  Setx0=off  InitialVoltage=0  SetiL0=off  InitialCurrent=0  Measurements=None  LoadType=constant I
      settings: SourceProductName=Simscape Electrical
  21 : powerlib/Measurements/Three-Phase V-I Measurement  VoltageMeasurement=phase-to-ground  SetLabelV=on  LabelV=V21  Vpu=off  VpuLL=off  CurrentMeasurement=no  SetLabelI=on  LabelI=I800  Ipu=off  Pbase=100e6  Vbase=24900  OutputType=Complex  PhasorSimulation=on  PSBequivalent=0
      settings: SourceProductName=Simscape Electrical
  21-22 10 : powerlib/Elements/Distributed Parameters Line  Phases=1  Frequency=60  Resistance=R_10(2,2)  Inductance=L_10(2,2)  Capacitance=C_10(2,2)  Length=525*ft2km  x1=[3345.99463574445;376.991118430775;-2.11628088240826]  x2=[3341.37996034713;376.991118430775;-2.11675110522689]  x3=[20.6052858605314;376.991118430775;0.427767335933522]  x4=[31.4925967537622;376.991118430775;-2.49340880492325]  x5=6.50871588399862e-07  V1=[2.049e+04;377;-2.115]  V2=[2.048e+04;377;-2.115]  I1=[33.62;377;-2.106]  I2=[35.2;377;-2.126]  nHarmo=1  Measurements=None
      settings: SourceProductName=Simscape Electrical
  21-23 2 : powerlib/Elements/Distributed Parameters Line  Phases=3  Frequency=60  Resistance=R_2  Inductance=L_2  Capacitance=C_2  Length=250*ft2km  x1=[494.38975347698 4006.40018891149 4050.73705232197;376.991118430775 376.991118430775 376.991118430775;-2.47552508488416 -0.338352122221564 -1.90046851498857]  x2=[496.272861993318 4003.97392325111 4049.99452748986;376.991118430775 376.991118430775 376.991118430775;-2.46802126679067 -0.338670530673969 -1.90076667258504]  x3=[43.6491359137779 79.2825543823426 27.4422588388052;376.991118430775 376.991118430775 376.991118430775;-2.55794930522497 2.11655322958947 1.04108422558873]  x4=[42.3520264065245 104.149007548009 51.0646445322742;376.991118430775 376.991118430775 376.991118430775;0.580998789894603 -0.842053808236458 -2.00755196140196]  x5=3.13537493203638e-07  V1=ones(3,3)  V2=ones(3,3)  I1=ones(3,3)  I2=ones(3,3)  nHarmo=1  Measurements=None
      settings: SourceProductName=Simscape Electrical
  22 : Subsystem
  22 Y Z : powerlib/Elements/Series RLC Load  LConnTagsString=a  RConnTagsString=__new0  NominalVoltage=1.0*2401.78  NominalFrequency=60  ActivePower=40e3*a  InductivePower=20e3*a  CapacitivePower=0  Setx0=off  InitialVoltage=0  SetiL0=off  InitialCurrent=0  Measurements=None  LoadType=constant Z
      settings: SourceProductName=Simscape Electrical
  23 : powerlib/Measurements/Three-Phase V-I Measurement  VoltageMeasurement=phase-to-ground  SetLabelV=on  LabelV=V23  Vpu=off  VpuLL=off  CurrentMeasurement=no  SetLabelI=on  LabelI=I800  Ipu=off  Pbase=100e6  Vbase=24900  OutputType=Complex  PhasorSimulation=on  PSBequivalent=0
      settings: SourceProductName=Simscape Electrical
  23-24 11 : powerlib/Elements/Distributed Parameters Line  Phases=1  Frequency=60  Resistance=R_11(3,3)  Inductance=L_11(3,3)  Capacitance=C_11(3,3)  Length=550*ft2km  x1=[3282.4290686518;376.991118430775;2.0735784648979]  x2=[3277.68677220532;376.991118430775;2.07308588320295]  x3=[20.2121850776963;376.991118430775;-1.6655963043086]  x4=[30.8921496519017;376.991118430775;1.69642609434551]  x5=6.8186547356176e-07  V1=[2.049e+04;377;-2.115]  V2=[2.048e+04;377;-2.115]  I1=[33.62;377;-2.106]  I2=[35.2;377;-2.126]  nHarmo=1  Measurements=None
      settings: SourceProductName=Simscape Electrical
  23-25 2 : powerlib/Elements/Distributed Parameters Line  Phases=3  Frequency=60  Resistance=R_2  Inductance=L_2  Capacitance=C_2  Length=275*ft2km  x1=[496.272861993318 4003.97392325111 4049.99452748986;376.991118430775 376.991118430775 376.991118430775;-2.46803308687569 -0.338680337621946 -1.90077643687671]  x2=[499.198521442782 4001.77784633656 4049.20411035162;376.991118430775 376.991118430775 376.991118430775;-2.46254731454081 -0.339046033120495 -1.90095480127127]  x3=[38.1382751948667 67.0429866563779 16.7379207855144;376.991118430775 376.991118430775 376.991118430775;-2.89644536376456 2.22132150087603 0.528155324552976]  x4=[36.9536255863911 93.4689764505432 38.1417012966944;376.991118430775 376.991118430775 376.991118430775;0.230351420309289 -0.743783595579957 -2.19189253782192]  x5=3.44891242524002e-07  V1=ones(3,3)  V2=ones(3,3)  I1=ones(3,3)  I2=ones(3,3)  nHarmo=1  Measurements=None
      settings: SourceProductName=Simscape Electrical
  24 : Subsystem
  24 Y PQ : powerlib/Elements/Series RLC Load  LConnTagsString=a  RConnTagsString=__new0  NominalVoltage=1.0*2401.78  NominalFrequency=60  ActivePower=40e3*a  InductivePower=20e3*a  CapacitivePower=0  Setx0=off  InitialVoltage=0  SetiL0=off  InitialCurrent=0  Measurements=None  LoadType=constant PQ
      settings: SourceProductName=Simscape Electrical
  25 : powerlib/Measurements/Three-Phase V-I Measurement  VoltageMeasurement=phase-to-ground  SetLabelV=on  LabelV=V25  Vpu=off  VpuLL=off  CurrentMeasurement=no  SetLabelI=on  LabelI=I800  Ipu=off  Pbase=100e6  Vbase=24900  OutputType=Complex  PhasorSimulation=on  PSBequivalent=0
      settings: SourceProductName=Simscape Electrical
  25-26 1 : powerlib/Elements/Distributed Parameters Line  Phases=2  Frequency=60  Resistance=R_7([1 3],[1 3])  Inductance=L_7([1 3],[1 3])  Capacitance=C_7([1 3],[1 3])  Length=350*ft2km  x1=[4011.65463779259 2266.70161003605;376.991118430775 376.991118430775;-0.556603764565277 1.01856342163721]  x2=[4010.45444908585 2265.32139710883;376.991118430775 376.991118430775;-0.556847393868056 1.01802863507945]  x3=[21.0223391052952 14.2221065485178;376.991118430775 376.991118430775;1.85496726645411 -2.69206770959397]  x4=[42.1701396143672 21.0245028156257;376.991118430775 376.991118430775;-0.895620064589545 0.645344940898273]  x5=4.29041749824869e-07  V1=ones(3,3)  V2=ones(3,3)  I1=ones(3,3)  I2=ones(3,3)  nHarmo=1  Measurements=None
      settings: SourceProductName=Simscape Electrical
  25-28 2 : powerlib/Elements/Distributed Parameters Line  Phases=3  Frequency=60  Resistance=R_2  Inductance=L_2  Capacitance=C_2  Length=200*ft2km  x1=[499.198521442782 4001.77784633656 4049.20411035162;376.991118430775 376.991118430775 376.991118430775;-2.46251185428574 -0.339016612276566 -1.90092550839626]  x2=[500.822385115609 4000.827558174 4048.82699490922;376.991118430775 376.991118430775 376.991118430775;-2.46052712326122 -0.339197795217479 -1.90097571924591]  x3=[25.080342040828 36.616211821853 9.13878022942413;376.991118430775 376.991118430775 376.991118430775;-3.08661562867689 2.22253812532276 -0.360005554806869]  x4=[24.0267624035187 63.7419122547267 25.3033074333558;376.991118430775 376.991118430775 376.991118430775;0.0229611397140362 -0.659355859620028 -2.27033920460248]  x5=2.50829994562911e-07  V1=ones(3,3)  V2=ones(3,3)  I1=ones(3,3)  I2=ones(3,3)  nHarmo=1  Measurements=None
      settings: SourceProductName=Simscape Electrical
  250 : powerlib/Measurements/Three-Phase V-I Measurement  VoltageMeasurement=phase-to-ground  SetLabelV=on  LabelV=V250  Vpu=off  VpuLL=off  CurrentMeasurement=no  SetLabelI=on  LabelI=I800  Ipu=off  Pbase=100e6  Vbase=24900  OutputType=Complex  PhasorSimulation=on  PSBequivalent=0
      settings: SourceProductName=Simscape Electrical
  250-251 : powerlib/Elements/Three-Phase Breaker  InitialState=open  SwitchA=on  SwitchB=on  SwitchC=on  SwitchTimes="[1/60  5/60]"  External=off  BreakerResistance=0.01  SnubberResistance=1e6  SnubberCapacitance=inf  Measurements=None
      settings: SourceProductName=Simscape Electrical
  26 : Subsystem
  26-27 7 : powerlib/Elements/Distributed Parameters Line  Phases=2  Frequency=60  Resistance=R_7([1 3],[1 3])  Inductance=L_7([1 3],[1 3])  Capacitance=C_7([1 3],[1 3])  Length=275*ft2km  x1=[4010.45444908585 2265.32139710883;376.991118430775 376.991118430775;-0.556818091178675 1.01806329470712]  x2=[4010.20749704044 2263.95335224525;376.991118430775 376.991118430775;-0.556978639956823 1.01828361680274]  x3=[5.61777532839839 17.921813873333;376.991118430775 376.991118430775;2.75167062500736 2.42446422393053]  x4=[29.6550964466308 18.283304919234;376.991118430775 376.991118430775;-0.525452111222503 -0.295089374042773]  x5=3.37104232005254e-07  V1=ones(3,3)  V2=ones(3,3)  I1=ones(3,3)  I2=ones(3,3)  nHarmo=1  Measurements=None
      settings: SourceProductName=Simscape Electrical
  26-31 1 : powerlib/Elements/Distributed Parameters Line  Phases=1  Frequency=60  Resistance=R_11(3,3)  Inductance=L_11(3,3)  Capacitance=C_11(3,3)  Length=225*ft2km  x1=[3277.91763971153;376.991118430775;2.07355283590532]  x2=[3275.97908174369;376.991118430775;2.07335122446513]  x3=[20.201489446981;376.991118430775;-1.66523907430257]  x4=[30.8730919978568;376.991118430775;1.6966810380654]  x5=2.78944966457084e-07  V1=[2.049e+04;377;-2.115]  V2=[2.048e+04;377;-2.115]  I1=[33.62;377;-2.106]  I2=[35.2;377;-2.126]  nHarmo=1  Measurements=None
      settings: SourceProductName=Simscape Electrical
  27 : Subsystem
  27-33 1 : powerlib/Elements/Distributed Parameters Line  Phases=1  Frequency=60  Resistance=R_9(1,1)  Inductance=L_9(1,1)  Capacitance=C_9(1,1)  Length=500*ft2km  x1=[3235.75541407692;376.991118430775;-0.0399677909730728]  x2=[3231.50501426449;376.991118430775;-0.0404156517963458]  x3=[19.9281207193047;376.991118430775;2.50411716702342]  x4=[30.457232653746;376.991118430775;-0.417072447057209]  x5=6.19877703237964e-07  V1=[2.049e+04;377;-2.115]  V2=[2.048e+04;377;-2.115]  I1=[33.62;377;-2.106]  I2=[35.2;377;-2.126]  nHarmo=1  Measurements=None
      settings: SourceProductName=Simscape Electrical
  28 : powerlib/Measurements/Three-Phase V-I Measurement  VoltageMeasurement=phase-to-ground  SetLabelV=on  LabelV=V28  Vpu=off  VpuLL=off  CurrentMeasurement=no  SetLabelI=on  LabelI=I800  Ipu=off  Pbase=100e6  Vbase=24900  OutputType=Complex  PhasorSimulation=on  PSBequivalent=0
      settings: SourceProductName=Simscape Electrical
  28 Y I : powerlib/Elements/Series RLC Load  LConnTagsString=a  RConnTagsString=__new0  NominalVoltage=1.0*2401.78  NominalFrequency=60  ActivePower=40e3*a  InductivePower=20e3*a  CapacitivePower=0  Setx0=off  InitialVoltage=0  SetiL0=off  InitialCurrent=0  Measurements=None  LoadType=constant I
      settings: SourceProductName=Simscape Electrical
  28-29 2 : powerlib/Elements/Distributed Parameters Line  Phases=3  Frequency=60  Resistance=R_2  Inductance=L_2  Capacitance=C_2  Length=300*ft2km  x1=[500.822385115609 4000.827558174 4048.82699490922;376.991118430775 376.991118430775 376.991118430775;-2.46057440360131 -0.339237023009385 -1.90101477641259]  x2=[501.595351749251 3999.85738615931 4048.53012753549;376.991118430775 376.991118430775 376.991118430775;-2.45762820099961 -0.339364778335102 -1.90113406810681]  x3=[14.9895301952397 19.7571145991462 2.075020014477;376.991118430775 376.991118430775 376.991118430775;-2.55546609138572 1.79240332528341 0.17699890779646]  x4=[13.6786880787288 43.7037698625883 24.9412052883421;376.991118430775 376.991118430775 376.991118430775;0.576865613640922 -0.732169136352526 -1.97391445581681]  x5=3.76244991844366e-07  V1=ones(3,3)  V2=ones(3,3)  I1=ones(3,3)  I2=ones(3,3)  nHarmo=1  Measurements=None
      settings: SourceProductName=Simscape Electrical
  29 : powerlib/Measurements/Three-Phase V-I Measurement  VoltageMeasurement=phase-to-ground  SetLabelV=on  LabelV=V29  Vpu=off  VpuLL=off  CurrentMeasurement=no  SetLabelI=on  LabelI=I800  Ipu=off  Pbase=100e6  Vbase=24900  OutputType=Complex  PhasorSimulation=on  PSBequivalent=0
      settings: SourceProductName=Simscape Electrical
  29 Y Z : powerlib/Elements/Series RLC Load  LConnTagsString=a  RConnTagsString=__new0  NominalVoltage=1.0*2401.78  NominalFrequency=60  ActivePower=40e3*a  InductivePower=20e3*a  CapacitivePower=0  Setx0=off  InitialVoltage=0  SetiL0=off  InitialCurrent=0  Measurements=None  LoadType=constant Z
      settings: SourceProductName=Simscape Electrical
  29-30 2 : powerlib/Elements/Distributed Parameters Line  Phases=3  Frequency=60  Resistance=R_2  Inductance=L_2  Capacitance=C_2  Length=350*ft2km  x1=[501.595351749251 3999.85738615931 4048.53012753549;376.991118430775 376.991118430775 376.991118430775;-2.45765184116966 -0.339384392231055 -1.90115359669015]  x2=[500.558701903993 3999.25660350185 4048.497332047;376.991118430775 376.991118430775 376.991118430775;-2.45421937729304 -0.339365357482504 -1.90134408165299]  x3=[15.2090517229734 16.483290028217 5.96323425180831;376.991118430775 376.991118430775 376.991118430775;-1.56663495981304 0.609232905354579 2.41708832337848]  x4=[14.4157222655976 24.2814154152088 26.7283481236546;376.991118430775 376.991118430775 376.991118430775;1.6459836911063 -0.923795507414959 -1.69381887328134]  x5=4.38952490485094e-07  V1=ones(3,3)  V2=ones(3,3)  I1=ones(3,3)  I2=ones(3,3)  nHarmo=1  Measurements=None
      settings: SourceProductName=Simscape Electrical
  3 : Subsystem
  3-4 11 : powerlib/Elements/Distributed Parameters Line  Phases=1  Frequency=60  Resistance=R_11(3,3)  Inductance=L_11(3,3)  Capacitance=C_11(3,3)  Length=200*ft2km  x1=[3355.99570274487;376.991118430775;2.0876641747894]  x2=[3354.23103300361;376.991118430775;2.08748489561966]  x3=[20.689769303733;376.991118430775;-1.65101004220151]  x4=[31.6163203822608;376.991118430775;1.71083057846377]  x5=2.47951081295186e-07  V1=[2.049e+04;377;-2.115]  V2=[2.048e+04;377;-2.115]  I1=[33.62;377;-2.106]  I2=[35.2;377;-2.126]  nHarmo=1  Measurements=None
      settings: SourceProductName=Simscape Electrical
  3-5 11 : powerlib/Elements/Distributed Parameters Line  Phases=1  Frequency=60  Resistance=R_11(3,3)  Inductance=L_11(3,3)  Capacitance=C_11(3,3)  Length=325*ft2km  x1=[3355.99570274487;376.991118430775;2.08760575269224]  x2=[3351.69910593112;376.991118430775;2.08716945372037]  x3=[33.573838270528;376.991118430775;-1.60022130955213]  x4=[44.5302086572559;376.991118430775;1.6850823477939]  x5=4.02920507104677e-07  V1=[2.049e+04;377;-2.115]  V2=[2.048e+04;377;-2.115]  I1=[33.62;377;-2.106]  I2=[35.2;377;-2.126]  nHarmo=1  Measurements=None
      settings: SourceProductName=Simscape Electrical
  "30 " : powerlib/Measurements/Three-Phase V-I Measurement  VoltageMeasurement=phase-to-ground  SetLabelV=on  LabelV=V30  Vpu=off  VpuLL=off  CurrentMeasurement=no  SetLabelI=on  LabelI=I800  Ipu=off  Pbase=100e6  Vbase=24900  OutputType=Complex  PhasorSimulation=on  PSBequivalent=0
      settings: SourceProductName=Simscape Electrical
  30 Y PQ : powerlib/Elements/Series RLC Load  LConnTagsString=a  RConnTagsString=__new0  NominalVoltage=1.0*2401.78  NominalFrequency=60  ActivePower=40e3*a  InductivePower=20e3*a  CapacitivePower=0  Setx0=off  InitialVoltage=0  SetiL0=off  InitialCurrent=0  Measurements=None  LoadType=constant PQ
      settings: SourceProductName=Simscape Electrical
  30-250 2 : powerlib/Elements/Distributed Parameters Line  Phases=3  Frequency=60  Resistance=R_2  Inductance=L_2  Capacitance=C_2  Length=200*ft2km  x1=[500.558701903993 3999.25660350185 4048.497332047;376.991118430775 376.991118430775 376.991118430775;-2.4541484567829 -0.339306515794647 -1.90128549590297]  x2=[500.558704141859 3999.25661581014 4048.49734439868;376.991118430775 376.991118430775 376.991118430775;-2.45414845857658 -0.339306517493266 -1.90128549723589]  x3=[0.65792178996951 14.9283337246899 11.933132132342;376.991118430775 376.991118430775 376.991118430775;-2.45424301746657 -0.339384972300633 -1.90136361094409]  x4=[0.657921791442997 14.9283337254943 11.9331321313309;376.991118430775 376.991118430775 376.991118430775;-2.45414845943649 -0.339306517423106 -1.90128549719426]  x5=2.50829994562911e-07  V1=ones(3,3)  V2=ones(3,3)  I1=ones(3,3)  I2=ones(3,3)  nHarmo=1  Measurements=None
      settings: SourceProductName=Simscape Electrical
  300 : powerlib/Measurements/Three-Phase V-I Measurement  VoltageMeasurement=phase-to-ground  SetLabelV=on  LabelV=V300  Vpu=off  VpuLL=off  CurrentMeasurement=no  SetLabelI=on  LabelI=I65  Ipu=off  Pbase=100e6  Vbase=24900  OutputType=Complex  PhasorSimulation=on  PSBequivalent=0
      settings: SourceProductName=Simscape Electrical
  300-1 : powerlib/Elements/Three-Phase Breaker  InitialState=open  SwitchA=off  SwitchB=off  SwitchC=off  SwitchTimes="[1/60  5/60]"  External=off  BreakerResistance=0.01  SnubberResistance=1e6  SnubberCapacitance=inf  Measurements=None
      settings: SourceProductName=Simscape Electrical
  31 : Subsystem
  31 Y PQ : powerlib/Elements/Series RLC Load  LConnTagsString=a  RConnTagsString=__new0  NominalVoltage=1.0*2401.78  NominalFrequency=60  ActivePower=20e3*a  InductivePower=10e3*a  CapacitivePower=0  Setx0=off  InitialVoltage=0  SetiL0=off  InitialCurrent=0  Measurements=None  LoadType=constant PQ
      settings: SourceProductName=Simscape Electrical
  31-32 1 : powerlib/Elements/Distributed Parameters Line  Phases=1  Frequency=60  Resistance=R_11(3,3)  Inductance=L_11(3,3)  Capacitance=C_11(3,3)  Length=300*ft2km  x1=[3275.97908174369;376.991118430775;2.07331617120684]  x2=[3274.68699699714;376.991118430775;2.0731816876914]  x3=[7.8029581610919;376.991118430775;-1.88302941674253]  x4=[18.2542915950686;376.991118430775;1.75697587902383]  x5=3.71926621942778e-07  V1=[2.049e+04;377;-2.115]  V2=[2.048e+04;377;-2.115]  I1=[33.62;377;-2.106]  I2=[35.2;377;-2.126]  nHarmo=1  Measurements=None
      settings: SourceProductName=Simscape Electrical
  32 : Subsystem
  32 Y PQ : powerlib/Elements/Series RLC Load  LConnTagsString=a  RConnTagsString=__new0  NominalVoltage=1.0*2401.78  NominalFrequency=60  ActivePower=20e3*a  InductivePower=10e3*a  CapacitivePower=0  Setx0=off  InitialVoltage=0  SetiL0=off  InitialCurrent=0  Measurements=None  LoadType=constant PQ
      settings: SourceProductName=Simscape Electrical
  33 : Subsystem
  33 Y I : powerlib/Elements/Series RLC Load  LConnTagsString=a  RConnTagsString=__new0  NominalVoltage=1.0*2401.78  NominalFrequency=60  ActivePower=40e3*a  InductivePower=20e3*a  CapacitivePower=0  Setx0=off  InitialVoltage=0  SetiL0=off  InitialCurrent=0  Measurements=None  LoadType=constant I
      settings: SourceProductName=Simscape Electrical
  34 : Subsystem
  34 Y Z : powerlib/Elements/Series RLC Load  LConnTagsString=a  RConnTagsString=__new0  NominalVoltage=1.0*2401.78  NominalFrequency=60  ActivePower=40e3*a  InductivePower=20e3*a  CapacitivePower=0  Setx0=off  InitialVoltage=0  SetiL0=off  InitialCurrent=0  Measurements=None  LoadType=constant Z
      settings: SourceProductName=Simscape Electrical
  34-15 11 : powerlib/Elements/Distributed Parameters Line  Phases=1  Frequency=60  Resistance=R_11(3,3)  Inductance=L_11(3,3)  Capacitance=C_11(3,3)  Length=100*ft2km  x1=[3310.76065547735;376.991118430775;2.07528698390433]  x2=[3309.45581098444;376.991118430775;2.07515271121131]  x3=[33.14167545582;376.991118430775;-1.61227292422966]  x4=[43.9562701080338;376.991118430775;1.67300443224042]  x5=1.23975540647593e-07  V1=[2.049e+04;377;-2.115]  V2=[2.048e+04;377;-2.115]  I1=[33.62;377;-2.106]  I2=[35.2;377;-2.126]  nHarmo=1  Measurements=None
      settings: SourceProductName=Simscape Electrical
  35 : powerlib/Measurements/Three-Phase V-I Measurement  VoltageMeasurement=phase-to-ground  SetLabelV=on  LabelV=V35  Vpu=off  VpuLL=off  CurrentMeasurement=no  SetLabelI=on  LabelI=I800  Ipu=off  Pbase=100e6  Vbase=24900  OutputType=Complex  PhasorSimulation=on  PSBequivalent=0
      settings: SourceProductName=Simscape Electrical
  35 D PQ : powerlib/Elements/Series RLC Load  LConnTagsString=a  RConnTagsString=__new0  NominalVoltage=1.0*4160  NominalFrequency=60  ActivePower=40e3*a  InductivePower=20e3*a  CapacitivePower=0  Setx0=off  InitialVoltage=0  SetiL0=off  InitialCurrent=0  Measurements=None  LoadType=constant I
      settings: SourceProductName=Simscape Electrical
  35-36 8 : powerlib/Elements/Distributed Parameters Line  Phases=2  Frequency=60  Resistance=R_8([1 2],[1 2])  Inductance=L_8([1 2],[1 2])  Capacitance=C_8([1 2],[1 2])  Length=650*ft2km  x1=[4005.1493980165 2352.6751194094;376.991118430775 376.991118430775;-2.63856955471155 -1.11394373273438]  x2=[4002.92480936606 2350.01265115801;376.991118430775 376.991118430775;-2.63902207891981 -1.11493555566952]  x3=[20.9813070558975 14.7588883491724;376.991118430775 376.991118430775;-0.226943846036592 1.45686649534731]  x4=[42.0932810590497 21.8129429368972;376.991118430775 376.991118430775;-2.97761748450232 -1.48843618981772]  x5=7.96791821103328e-07  V1=ones(3,3)  V2=ones(3,3)  I1=ones(3,3)  I2=ones(3,3)  nHarmo=1  Measurements=None
      settings: SourceProductName=Simscape Electrical
  35-40 1 : powerlib/Elements/Distributed Parameters Line  Phases=3  Frequency=60  Resistance=R_1  Inductance=L_1  Capacitance=C_1  Length=250*ft2km  x1=[381.136339799871 4017.58988064936 4025.47842825818;376.991118430775 376.991118430775 376.991118430775;1.80511471029563 -2.42167330013699 2.27595618191813]  x2=[381.652314983168 4012.75291737624 4020.42951070777;376.991118430775 376.991118430775 376.991118430775;1.80560445779725 -2.42228318013172 2.27508704745884]  x3=[6.00861530839697 168.485296291642 159.914581923679;376.991118430775 376.991118430775 376.991118430775;1.02563100448618 0.0716413344642967 -1.4582971231685]  x4=[5.34233583728707 193.23442490146 180.079184777451;376.991118430775 376.991118430775 376.991118430775;-2.24828611869194 -2.97619180753216 1.7568699762705]  x5=3.13537493203638e-07  V1=ones(3,3)  V2=ones(3,3)  I1=ones(3,3)  I2=ones(3,3)  nHarmo=1  Measurements=None
      settings: SourceProductName=Simscape Electrical
  36 : Subsystem
  36-37 9 : powerlib/Elements/Distributed Parameters Line  Phases=1  Frequency=60  Resistance=R_9(1,1)  Inductance=L_9(1,1)  Capacitance=C_9(1,1)  Length=300*ft2km  x1=[3229.66139179001;376.991118430775;-0.0378136444169964]  x2=[3227.11467322558;376.991118430775;-0.038082495712426]  x3=[19.9041371159127;376.991118430775;2.50655535194466]  x4=[30.4173822298935;376.991118430775;-0.414737644054704]  x5=3.71926621942778e-07  V1=[2.049e+04;377;-2.115]  V2=[2.048e+04;377;-2.115]  I1=[33.62;377;-2.106]  I2=[35.2;377;-2.126]  nHarmo=1  Measurements=None
      settings: SourceProductName=Simscape Electrical
  36-38 10 : powerlib/Elements/Distributed Parameters Line  Phases=1  Frequency=60  Resistance=R_10(2,2)  Inductance=L_10(2,2)  Capacitance=C_10(2,2)  Length=250*ft2km  x1=[3334.07277976194;376.991118430775;-2.11815142863613]  x2=[3331.88210055984;376.991118430775;-2.11837542128896]  x3=[20.5453780192118;376.991118430775;0.426199608567581]  x4=[31.399267778862;376.991118430775;-2.49504711725883]  x5=3.09938851618982e-07  V1=[2.049e+04;377;-2.115]  V2=[2.048e+04;377;-2.115]  I1=[33.62;377;-2.106]  I2=[35.2;377;-2.126]  nHarmo=1  Measurements=None
      settings: SourceProductName=Simscape Electrical
  37 : Subsystem
  37 Y Z : powerlib/Elements/Series RLC Load  LConnTagsString=a  RConnTagsString=__new0  NominalVoltage=1.0*2401.78  NominalFrequency=60  ActivePower=40e3*a  InductivePower=20e3*a  CapacitivePower=0  Setx0=off  InitialVoltage=0  SetiL0=off  InitialCurrent=0  Measurements=None  LoadType=constant Z
      settings: SourceProductName=Simscape Electrical
  38 : Subsystem
  38 Y I : powerlib/Elements/Series RLC Load  LConnTagsString=a  RConnTagsString=__new0  NominalVoltage=1.0*2401.78  NominalFrequency=60  ActivePower=20e3*a  InductivePower=10e3*a  CapacitivePower=0  Setx0=off  InitialVoltage=0  SetiL0=off  InitialCurrent=0  Measurements=None  LoadType=constant I
      settings: SourceProductName=Simscape Electrical
  38-39 10 : powerlib/Elements/Distributed Parameters Line  Phases=1  Frequency=60  Resistance=R_10(2,2)  Inductance=L_10(2,2)  Capacitance=C_10(2,2)  Length=325*ft2km  x1=[3331.88210055984;376.991118430775;-2.11841047454725]  x2=[3330.45850290638;376.991118430775;-2.11855616110939]  x3=[7.93567766815194;376.991118430775;0.208401523438884]  x4=[18.565058452383;376.991118430775;-2.43476226297961]  x5=4.02920507104677e-07  V1=[2.049e+04;377;-2.115]  V2=[2.048e+04;377;-2.115]  I1=[33.62;377;-2.106]  I2=[35.2;377;-2.126]  nHarmo=1  Measurements=None
      settings: SourceProductName=Simscape Electrical
  39 : Subsystem
  39 Y PQ : powerlib/Elements/Series RLC Load  LConnTagsString=a  RConnTagsString=__new0  NominalVoltage=1.0*2401.78  NominalFrequency=60  ActivePower=20e3*a  InductivePower=10e3*a  CapacitivePower=0  Setx0=off  InitialVoltage=0  SetiL0=off  InitialCurrent=0  Measurements=None  LoadType=constant PQ
      settings: SourceProductName=Simscape Electrical
  4 : Subsystem
  40 : powerlib/Measurements/Three-Phase V-I Measurement  VoltageMeasurement=phase-to-ground  SetLabelV=on  LabelV=V40  Vpu=off  VpuLL=off  CurrentMeasurement=no  SetLabelI=on  LabelI=I800  Ipu=off  Pbase=100e6  Vbase=24900  OutputType=Complex  PhasorSimulation=on  PSBequivalent=0
      settings: SourceProductName=Simscape Electrical
  40-41 11 : powerlib/Elements/Distributed Parameters Line  Phases=1  Frequency=60  Resistance=R_11(3,3)  Inductance=L_11(3,3)  Capacitance=C_11(3,3)  Length=325*ft2km  x1=[3281.98720528819;376.991118430775;2.07257203125346]  x2=[3280.5849260196;376.991118430775;2.07242634468541]  x3=[7.81684075509191;376.991118430775;-1.88380125733379]  x4=[18.2870467925264;376.991118430775;1.75622025665551]  x5=4.02920507104677e-07  V1=[2.049e+04;377;-2.115]  V2=[2.048e+04;377;-2.115]  I1=[33.62;377;-2.106]  I2=[35.2;377;-2.126]  nHarmo=1  Measurements=None
      settings: SourceProductName=Simscape Electrical
  40-42 1 : powerlib/Elements/Distributed Parameters Line  Phases=3  Frequency=60  Resistance=R_1  Inductance=L_1  Capacitance=C_1  Length=250*ft2km  x1=[381.652314983168 4012.75291737624 4020.42951070777;376.991118430775 376.991118430775 376.991118430775;1.80560445779725 -2.42228318013172 2.27508704745884]  x2=[382.56760243676 4007.89744646488 4015.68619500456;376.991118430775 376.991118430775 376.991118430775;1.80768812111448 -2.4228822643485 2.27425627131396]  x3=[12.9685979041758 168.444867983133 150.444970069188;376.991118430775 376.991118430775 376.991118430775;1.35089037799101 0.0612535934526647 -1.45349539415523]  x4=[12.0747300622017 193.008199757821 170.677086681775;376.991118430775 376.991118430775 376.991118430775;-1.82732027947756 -2.98537206487155 1.76498400075355]  x5=3.13537493203638e-07  V1=ones(3,3)  V2=ones(3,3)  I1=ones(3,3)  I2=ones(3,3)  nHarmo=1  Measurements=None
      settings: SourceProductName=Simscape Electrical
  41 : Subsystem
  41 Y PQ : powerlib/Elements/Series RLC Load  LConnTagsString=a  RConnTagsString=__new0  NominalVoltage=1.0*2401.78  NominalFrequency=60  ActivePower=20e3*a  InductivePower=10e3*a  CapacitivePower=0  Setx0=off  InitialVoltage=0  SetiL0=off  InitialCurrent=0  Measurements=None  LoadType=constant PQ
      settings: SourceProductName=Simscape Electrical
  4160 V swing : powerlib/Electrical Sources/Three-Phase Source  InternalConnection=Yg  VoltagePhases=on  Voltage=120e3  PhaseAngle=0  Voltage_phases=[1.0 1.0 1.0]*4160/sqrt(3)  PhaseAngles_phases=[0 -120 120 ]  Frequency=60  NonIdealSource=off  SpecifyImpedance=on  Resistance=.0001  Inductance=16.58e-3  ShortCircuitLevel=10e6  BaseVoltage=4160  XRratio=4.67e4  BusType=swing  Pref=0  Qref=0  Prefabc=[4e6/3 4e6/3 4e6/3]  Qrefabc=[0 0 0]  Qmin="[-inf  -inf -inf]"  Qmax="[inf  inf inf]"
      settings: SourceProductName=Simscape Electrical
  42 : powerlib/Measurements/Three-Phase V-I Measurement  VoltageMeasurement=phase-to-ground  SetLabelV=on  LabelV=V42  Vpu=off  VpuLL=off  CurrentMeasurement=no  SetLabelI=on  LabelI=I800  Ipu=off  Pbase=100e6  Vbase=24900  OutputType=Complex  PhasorSimulation=on  PSBequivalent=0
      settings: SourceProductName=Simscape Electrical
  42 Y PQ : powerlib/Elements/Series RLC Load  LConnTagsString=a  RConnTagsString=__new0  NominalVoltage=1.0*2401.78  NominalFrequency=60  ActivePower=20e3*a  InductivePower=10e3*a  CapacitivePower=0  Setx0=off  InitialVoltage=0  SetiL0=off  InitialCurrent=0  Measurements=None  LoadType=constant PQ
      settings: SourceProductName=Simscape Electrical
  42-43 10 : powerlib/Elements/Distributed Parameters Line  Phases=1  Frequency=60  Resistance=R_10(2,2)  Inductance=L_10(2,2)  Capacitance=C_10(2,2)  Length=500*ft2km  x1=[3327.8139835034;376.991118430775;-2.11916004176177]  x2=[3323.44265806914;376.991118430775;-2.11960790257837]  x3=[20.4950839236898;376.991118430775;0.424924910168314]  x4=[31.3237533866193;376.991118430775;-2.49626470166047]  x5=6.19877703237964e-07  V1=[2.049e+04;377;-2.115]  V2=[2.048e+04;377;-2.115]  I1=[33.62;377;-2.106]  I2=[35.2;377;-2.126]  nHarmo=1  Measurements=None
      settings: SourceProductName=Simscape Electrical
  42-44 1 : powerlib/Elements/Distributed Parameters Line  Phases=3  Frequency=60  Resistance=R_1  Inductance=L_1  Capacitance=C_1  Length=200*ft2km  x1=[382.56760243676 4007.89744646488 4015.68619500456;376.991118430775 376.991118430775 376.991118430775;1.80771176128452 -2.42286265045255 2.2742757998973]  x2=[382.407419313175 4004.49225833245 4012.09095847134;376.991118430775 376.991118430775 376.991118430775;1.8082247936735 -2.42325058906558 2.27363475079142]  x3=[3.53827512931875 144.182284988192 142.839249128642;376.991118430775 376.991118430775 376.991118430775;2.74935600526469 0.0183497993005213 -1.44782528979466]  x4=[3.05648973752037 168.162550786504 163.146301003146;376.991118430775 376.991118430775 376.991118430775;-0.123065267575427 -3.00839352107728 1.77335314503737]  x5=2.50829994562911e-07  V1=ones(3,3)  V2=ones(3,3)  I1=ones(3,3)  I2=ones(3,3)  nHarmo=1  Measurements=None
      settings: SourceProductName=Simscape Electrical
  43 : Subsystem
  43 Y Z : powerlib/Elements/Series RLC Load  LConnTagsString=a  RConnTagsString=__new0  NominalVoltage=1.0*2401.78  NominalFrequency=60  ActivePower=40e3*a  InductivePower=20e3*a  CapacitivePower=0  Setx0=off  InitialVoltage=0  SetiL0=off  InitialCurrent=0  Measurements=None  LoadType=constant Z
      settings: SourceProductName=Simscape Electrical
  44 : powerlib/Measurements/Three-Phase V-I Measurement  VoltageMeasurement=phase-to-ground  SetLabelV=on  LabelV=V44  Vpu=off  VpuLL=off  CurrentMeasurement=no  SetLabelI=on  LabelI=I800  Ipu=off  Pbase=100e6  Vbase=24900  OutputType=Complex  PhasorSimulation=on  PSBequivalent=0
      settings: SourceProductName=Simscape Electrical
  44-45 9 : powerlib/Elements/Distributed Parameters Line  Phases=1  Frequency=60  Resistance=R_9(1,1)  Inductance=L_9(1,1)  Capacitance=C_9(1,1)  Length=200*ft2km  x1=[3219.33633750241;376.991118430775;-0.0390305340520873]  x2=[3217.64386387494;376.991118430775;-0.0392097554584136]  x3=[19.842147200141;376.991118430775;2.50539838252655]  x4=[30.32352636098;376.991118430775;-0.415879732351309]  x5=2.47951081295186e-07  V1=[2.049e+04;377;-2.115]  V2=[2.048e+04;377;-2.115]  I1=[33.62;377;-2.106]  I2=[35.2;377;-2.126]  nHarmo=1  Measurements=None
      settings: SourceProductName=Simscape Electrical
  44-47 1 : powerlib/Elements/Distributed Parameters Line  Phases=3  Frequency=60  Resistance=R_1  Inductance=L_1  Capacitance=C_1  Length=250*ft2km  x1=[382.407419313175 4004.49225833245 4012.09095847134;376.991118430775 376.991118430775 376.991118430775;1.80820115350345 -2.42327020296153 2.27361522220808]  x2=[382.82008824509 4000.65643860261 4007.62413603212;376.991118430775 376.991118430775 376.991118430775;1.80552668383886 -2.42377236618447 2.27294726439942]  x3=[11.0295278884369 132.098040362088 134.617469547841;376.991118430775 376.991118430775 376.991118430775;-0.538360893166279 0.0718164704648604 -1.53806070635489]  x4=[11.7548498432947 156.988973729888 153.851434642435;376.991118430775 376.991118430775 376.991118430775;2.54202730376297 -2.95490862680763 1.69905175880838]  x5=3.13537493203638e-07  V1=ones(3,3)  V2=ones(3,3)  I1=ones(3,3)  I2=ones(3,3)  nHarmo=1  Measurements=None
      settings: SourceProductName=Simscape Electrical
  45 : Subsystem
  45 Y I : powerlib/Elements/Series RLC Load  LConnTagsString=a  RConnTagsString=__new0  NominalVoltage=1.0*2401.78  NominalFrequency=60  ActivePower=20e3*a  InductivePower=10e3*a  CapacitivePower=0  Setx0=off  InitialVoltage=0  SetiL0=off  InitialCurrent=0  Measurements=None  LoadType=constant I
      settings: SourceProductName=Simscape Electrical
  45-46 9 : powerlib/Elements/Distributed Parameters Line  Phases=1  Frequency=60  Resistance=R_9(1,1)  Inductance=L_9(1,1)  Capacitance=C_9(1,1)  Length=300*ft2km  x1=[3217.64386387494;376.991118430775;-0.0392564931361404]  x2=[3216.3747872295;376.991118430775;-0.0393909766517211]  x3=[7.66401118625679;376.991118430775;2.28758322654961]  x4=[17.9292381837257;376.991118430775;-0.355596784182056]  x5=3.71926621942778e-07  V1=[2.049e+04;377;-2.115]  V2=[2.048e+04;377;-2.115]  I1=[33.62;377;-2.106]  I2=[35.2;377;-2.126]  nHarmo=1  Measurements=None
      settings: SourceProductName=Simscape Electrical
  450 : powerlib/Measurements/Three-Phase V-I Measurement  VoltageMeasurement=phase-to-ground  SetLabelV=on  LabelV=V450  Vpu=off  VpuLL=off  CurrentMeasurement=no  SetLabelI=on  LabelI=I65  Ipu=off  Pbase=100e6  Vbase=24900  OutputType=Complex  PhasorSimulation=on  PSBequivalent=0
      settings: SourceProductName=Simscape Electrical
  450-451 : powerlib/Elements/Three-Phase Breaker  InitialState=open  SwitchA=off  SwitchB=off  SwitchC=off  SwitchTimes="[1/60  5/60]"  External=off  BreakerResistance=0.01  SnubberResistance=1e6  SnubberCapacitance=inf  Measurements=None
      settings: SourceProductName=Simscape Electrical
  46 : Subsystem
  46 Y PQ : powerlib/Elements/Series RLC Load  LConnTagsString=a  RConnTagsString=__new0  NominalVoltage=1.0*2401.78  NominalFrequency=60  ActivePower=20e3*a  InductivePower=10e3*a  CapacitivePower=0  Setx0=off  InitialVoltage=0  SetiL0=off  InitialCurrent=0  Measurements=None  LoadType=constant PQ
      settings: SourceProductName=Simscape Electrical
  47 : powerlib/Measurements/Three-Phase V-I Measurement  VoltageMeasurement=phase-to-ground  SetLabelV=on  LabelV=V47  Vpu=off  VpuLL=off  CurrentMeasurement=no  SetLabelI=on  LabelI=I800  Ipu=off  Pbase=100e6  Vbase=24900  OutputType=Complex  PhasorSimulation=on  PSBequivalent=0
      settings: SourceProductName=Simscape Electrical
  47 Y I : powerlib/Elements/Three-Phase Series RLC Load  LConnTagsString=A|B|C  Configuration=Y (grounded)  NominalVoltage=120e3  Vabc=[ 1.0 1.0 1.0]*2401.78  Vabcp=[1e3 1e3 1e3]  NominalFrequency=60  UnbalancedPower=on  ActivePower=1e+006  InductivePower=0  CapacitivePower=0  Pabc=[35 35 35 ]*1e3*a  QLabc=[25 25 25 ]*1e3*a  QCabc=[0 0 0]  Pabcp=[10e3 9e3 11e3]  QLabcp=[100 90 110]  QCabcp=[100 90 110]  Measurements=None  LoadType=constant I
      settings: SourceProductName=Simscape Electrical
  47-48 4 : powerlib/Elements/Distributed Parameters Line  Phases=3  Frequency=60  Resistance=R_4  Inductance=L_4  Capacitance=C_4  Length=150*ft2km  x1=[353.205602428726 3975.3259044728 4032.99362637294;376.991118430775 376.991118430775 376.991118430775;0.301588362021023 -0.249192536085936 -1.81272340576746]  x2=[353.738095583081 3973.81878949399 4031.6058037247;376.991118430775 376.991118430775 376.991118430775;0.302208505037744 -0.24943562415048 -1.81290727114106]  x3=[10.2343736558157 73.0834923310974 75.2123885835248;376.991118430775 376.991118430775 376.991118430775;-0.464366994756412 2.2142804589805 0.643723471264721]  x4=[9.58653809340675 92.5071734823169 100.348804061354;376.991118430775 376.991118430775 376.991118430775;2.6099633627654 -0.767773198009124 -2.30690972800166]  x5=1.88122495922183e-07  V1=ones(3,3)  V2=ones(3,3)  I1=ones(3,3)  I2=ones(3,3)  nHarmo=1  Measurements=None
      settings: SourceProductName=Simscape Electrical
  47-49 4 : powerlib/Elements/Distributed Parameters Line  Phases=3  Frequency=60  Resistance=R_4  Inductance=L_4  Capacitance=C_4  Length=250*ft2km  x1=[353.738095583081 3973.81878949399 4031.6058037247;376.991118430775 376.991118430775 376.991118430775;0.302161224697651 -0.249474681317157 -1.81294649893297]  x2=[354.627065217543 3972.22776461026 4030.10685196723;376.991118430775 376.991118430775 376.991118430775;0.303154357020247 -0.24974159017751 -1.8131565000501]  x3=[10.1920937475295 43.5003542685413 45.250173771221;376.991118430775 376.991118430775 376.991118430775;-0.47672964606504 2.17491522645697 0.600706557061453]  x4=[9.55219630182743 63.0615073927143 70.6153412522447;376.991118430775 376.991118430775 376.991118430775;2.59630733029669 -0.720123101139686 -2.25346623652161]  x5=3.13537493203638e-07  V1=ones(3,3)  V2=ones(3,3)  I1=ones(3,3)  I2=ones(3,3)  nHarmo=1  Measurements=None
      settings: SourceProductName=Simscape Electrical
  48 : powerlib/Measurements/Three-Phase V-I Measurement  VoltageMeasurement=phase-to-ground  SetLabelV=on  LabelV=V48  Vpu=off  VpuLL=off  CurrentMeasurement=no  SetLabelI=on  LabelI=I800  Ipu=off  Pbase=100e6  Vbase=24900  OutputType=Complex  PhasorSimulation=on  PSBequivalent=0
      settings: SourceProductName=Simscape Electrical
  48 Y Z : powerlib/Elements/Three-Phase Series RLC Load  LConnTagsString=A|B|C  Configuration=Y (grounded)  NominalVoltage=120e3  Vabc=[ 1.0 1.0 1.0]*2401.78  Vabcp=[1e3 1e3 1e3]  NominalFrequency=60  UnbalancedPower=on  ActivePower=1e+006  InductivePower=0  CapacitivePower=0  Pabc=[70 70 70]*1e3*a  QLabc=[50 50 50]*1e3*a  QCabc=[0 0 0]  Pabcp=[10e3 9e3 11e3]  QLabcp=[100 90 110]  QCabcp=[100 90 110]  Measurements=None  LoadType=constant Z
      settings: SourceProductName=Simscape Electrical
  49 : powerlib/Measurements/Three-Phase V-I Measurement  VoltageMeasurement=phase-to-ground  SetLabelV=on  LabelV=V49  Vpu=off  VpuLL=off  CurrentMeasurement=no  SetLabelI=on  LabelI=I800  Ipu=off  Pbase=100e6  Vbase=24900  OutputType=Complex  PhasorSimulation=on  PSBequivalent=0
      settings: SourceProductName=Simscape Electrical
  49 Y PQ : powerlib/Elements/Three-Phase Series RLC Load  LConnTagsString=A|B|C  Configuration=Y (grounded)  NominalVoltage=120e3  Vabc=[ 1.0 1.0 1.0]*2401.78  Vabcp=[1e3 1e3 1e3]  NominalFrequency=60  UnbalancedPower=on  ActivePower=1e+006  InductivePower=0  CapacitivePower=0  Pabc=[35 70 35]*1e3*a  QLabc=[25 50 20]*1e3*a  QCabc=[0 0 0]  Pabcp=[10e3 9e3 11e3]  QLabcp=[100 90 110]  QCabcp=[100 90 110]  Measurements=None  LoadType=constant PQ
      settings: SourceProductName=Simscape Electrical
  49-50 4 : powerlib/Elements/Distributed Parameters Line  Phases=3  Frequency=60  Resistance=R_4  Inductance=L_4  Capacitance=C_4  Length=250*ft2km  x1=[354.627065217543 3972.22776461026 4030.10685196723;376.991118430775 376.991118430775 376.991118430775;0.303154357020247 -0.24974159017751 -1.8131565000501]  x2=[355.106752911841 3971.47399639136 4029.97237075623;376.991118430775 376.991118430775 376.991118430775;0.299964113119355 -0.249790694491117 -1.81325201684314]  x3=[12.3625718290342 17.020634778059 2.80864866486195;376.991118430775 376.991118430775 376.991118430775;-2.03119412364892 1.41418968057324 -2.75730833377225]  x4=[13.0240130568246 30.2012362908529 28.5297769439255;376.991118430775 376.991118430775 376.991118430775;1.05855242088239 -0.845562623160587 -1.73343272700803]  x5=3.13537493203638e-07  V1=ones(3,3)  V2=ones(3,3)  I1=ones(3,3)  I2=ones(3,3)  nHarmo=1  Measurements=None
      settings: SourceProductName=Simscape Electrical
  4Y PQ : powerlib/Elements/Series RLC Load  LConnTagsString=a  RConnTagsString=__new0  NominalVoltage=1.0*2401.78  NominalFrequency=60  ActivePower=40e3*a  InductivePower=20e3*a  CapacitivePower=0  Setx0=off  InitialVoltage=0  SetiL0=off  InitialCurrent=0  Measurements=None  LoadType=constant PQ
      settings: SourceProductName=Simscape Electrical
  5 : Subsystem
  5 Y I : powerlib/Elements/Series RLC Load  LConnTagsString=a  RConnTagsString=__new0  NominalVoltage=1.0*2401.78  NominalFrequency=60  ActivePower=20e3*a  InductivePower=10e3*a  CapacitivePower=0  Setx0=off  InitialVoltage=0  SetiL0=off  InitialCurrent=0  Measurements=None  LoadType=constant I
      settings: SourceProductName=Simscape Electrical
  5-6 11 : powerlib/Elements/Distributed Parameters Line  Phases=1  Frequency=60  Resistance=R_11(3,3)  Inductance=L_11(3,3)  Capacitance=C_11(3,3)  Length=250*ft2km  x1=[3351.69910593112;376.991118430775;2.08720450697867]  x2=[3349.49637014091;376.991118430775;2.08698043613051]  x3=[20.6597627221231;376.991118430775;-1.65154076739136]  x4=[31.5712957352062;376.991118430775;1.71032569957829]  x5=3.09938851618982e-07  V1=[2.049e+04;377;-2.115]  V2=[2.048e+04;377;-2.115]  I1=[33.62;377;-2.106]  I2=[35.2;377;-2.126]  nHarmo=1  Measurements=None
      settings: SourceProductName=Simscape Electrical
  50 : powerlib/Measurements/Three-Phase V-I Measurement  VoltageMeasurement=phase-to-ground  SetLabelV=on  LabelV=V50  Vpu=off  VpuLL=off  CurrentMeasurement=no  SetLabelI=on  LabelI=I800  Ipu=off  Pbase=100e6  Vbase=24900  OutputType=Complex  PhasorSimulation=on  PSBequivalent=0
      settings: SourceProductName=Simscape Electrical
  50 Y PQ : powerlib/Elements/Series RLC Load  LConnTagsString=a  RConnTagsString=__new0  NominalVoltage=1.0*2401.78  NominalFrequency=60  ActivePower=40e3*a  InductivePower=20e3*a  CapacitivePower=0  Setx0=off  InitialVoltage=0  SetiL0=off  InitialCurrent=0  Measurements=None  LoadType=constant PQ
      settings: SourceProductName=Simscape Electrical
  50-51 4 : powerlib/Elements/Distributed Parameters Line  Phases=3  Frequency=60  Resistance=R_4  Inductance=L_4  Capacitance=C_4  Length=250*ft2km  x1=[355.106752911841 3971.47399639136 4029.97237075623;376.991118430775 376.991118430775 376.991118430775;0.299964113119355 -0.249790694491117 -1.81325201684314]  x2=[354.445169359047 3971.266208225 4029.93499702574;376.991118430775 376.991118430775 376.991118430775;0.299206077513577 -0.249857369496164 -1.81324309578913]  x3=[7.05433729211781 3.56381840973803 15.5795558058854;376.991118430775 376.991118430775 376.991118430775;2.59035787913497 0.464439076844732 -1.70594627617497]  x4=[7.7012922191929 20.8499422409075 14.6908654658384;376.991118430775 376.991118430775 376.991118430775;-0.460069240342314 -0.362082070010655 -1.92716821806741]  x5=3.13537493203638e-07  V1=ones(3,3)  V2=ones(3,3)  I1=ones(3,3)  I2=ones(3,3)  nHarmo=1  Measurements=None
      settings: SourceProductName=Simscape Electrical
  51 : powerlib/Measurements/Three-Phase V-I Measurement  VoltageMeasurement=phase-to-ground  SetLabelV=on  LabelV=V51  Vpu=off  VpuLL=off  CurrentMeasurement=no  SetLabelI=on  LabelI=I800  Ipu=off  Pbase=100e6  Vbase=24900  OutputType=Complex  PhasorSimulation=on  PSBequivalent=0
      settings: SourceProductName=Simscape Electrical
  51 Y PQ : powerlib/Elements/Series RLC Load  LConnTagsString=a  RConnTagsString=__new0  NominalVoltage=1.0*2401.78  NominalFrequency=60  ActivePower=20e3*a  InductivePower=10e3*a  CapacitivePower=0  Setx0=off  InitialVoltage=0  SetiL0=off  InitialCurrent=0  Measurements=None  LoadType=constant PQ
      settings: SourceProductName=Simscape Electrical
  51-151 4 : powerlib/Elements/Distributed Parameters Line  Phases=3  Frequency=60  Resistance=R_4  Inductance=L_4  Capacitance=C_4  Length=500*ft2km  x1=[354.445169359047 3971.266208225 4029.93499702574;376.991118430775 376.991118430775 376.991118430775;0.299087876663344 -0.249955012412857 -1.8133411652689]  x2=[354.445181005013 3971.26628822914 4029.9350771673;376.991118430775 376.991118430775 376.991118430775;0.299087856046001 -0.24995502186148 -1.81334117657001]  x3=[0.465841342590965 11.7050080709569 15.0420976895419;376.991118430775 376.991118430775 376.991118430775;0.298819805236217 -0.250157036219535 -1.81354133224162]  x4=[0.465866585449303 11.7050732101689 15.0421359338811;376.991118430775 376.991118430775 376.991118430775;0.299119512036717 -0.249948288634372 -1.81333715412465]  x5=6.27074986407277e-07  V1=ones(3,3)  V2=ones(3,3)  I1=ones(3,3)  I2=ones(3,3)  nHarmo=1  Measurements=None
      settings: SourceProductName=Simscape Electrical
  52 : powerlib/Measurements/Three-Phase V-I Measurement  VoltageMeasurement=phase-to-ground  SetLabelV=on  LabelV=V52  Vpu=off  VpuLL=off  CurrentMeasurement=no  SetLabelI=on  LabelI=I65  Ipu=off  Pbase=100e6  Vbase=24900  OutputType=Complex  PhasorSimulation=on  PSBequivalent=0
      settings: SourceProductName=Simscape Electrical
  52 Y PQ : powerlib/Elements/Series RLC Load  LConnTagsString=a  RConnTagsString=__new0  NominalVoltage=1.0*2401.78  NominalFrequency=60  ActivePower=40e3*a  InductivePower=20e3*a  CapacitivePower=0  Setx0=off  InitialVoltage=0  SetiL0=off  InitialCurrent=0  Measurements=None  LoadType=constant PQ
      settings: SourceProductName=Simscape Electrical
  52-53 1 : powerlib/Elements/Distributed Parameters Line  Phases=3  Frequency=60  Resistance=R_1  Inductance=L_1  Capacitance=C_1  Length=200*ft2km  x1=[387.990472092363 4040.29436483784 4040.67700374777;376.991118430775 376.991118430775 376.991118430775;1.78466066536762 -2.42004214182878 2.2757747011722]  x2=[386.566822000311 4033.19969990484 4034.06103349489;376.991118430775 376.991118430775 376.991118430775;1.78992569153632 -2.42194088697507 2.2728399061029]  x3=[32.3626571600528 420.438788842689 457.400851388472;376.991118430775 376.991118430775 376.991118430775;2.7651240657251 0.469481687833197 -0.967195319310226]  x4=[31.8049970256746 449.692718180079 481.088740039824;376.991118430775 376.991118430775 376.991118430775;-0.34991964963013 -2.65546002318535 2.17933006222332]  x5=2.50829994562911e-07  V1=ones(3,3)  V2=ones(3,3)  I1=ones(3,3)  I2=ones(3,3)  nHarmo=1  Measurements=None
      settings: SourceProductName=Simscape Electrical
  53 : powerlib/Measurements/Three-Phase V-I Measurement  VoltageMeasurement=phase-to-ground  SetLabelV=on  LabelV=V53  Vpu=off  VpuLL=off  CurrentMeasurement=no  SetLabelI=on  LabelI=I65  Ipu=off  Pbase=100e6  Vbase=24900  OutputType=Complex  PhasorSimulation=on  PSBequivalent=0
      settings: SourceProductName=Simscape Electrical
  53 Y PQ : powerlib/Elements/Series RLC Load  LConnTagsString=a  RConnTagsString=__new0  NominalVoltage=1.0*2401.78  NominalFrequency=60  ActivePower=40e3*a  InductivePower=20e3*a  CapacitivePower=0  Setx0=off  InitialVoltage=0  SetiL0=off  InitialCurrent=0  Measurements=None  LoadType=constant PQ
      settings: SourceProductName=Simscape Electrical
  53-54 1 : powerlib/Elements/Distributed Parameters Line  Phases=3  Frequency=60  Resistance=R_1  Inductance=L_1  Capacitance=C_1  Length=125*ft2km  x1=[386.566822000311 4033.19969990484 4034.06103349489;376.991118430775 376.991118430775 376.991118430775;1.78996115179139 -2.42191146613114 2.27286919897791]  x2=[386.001754491217 4028.98439798237 4029.95524089406;376.991118430775 376.991118430775 376.991118430775;1.79162948600345 -2.42310965991927 2.2710976704245]  x3=[17.926540626558 412.57245944311 443.996095452947;376.991118430775 376.991118430775 376.991118430775;2.86688566726082 0.498114783963688 -0.982361836263193]  x4=[17.4673358970817 441.984800794537 467.622150312356;376.991118430775 376.991118430775 376.991118430775;-0.223519125654147 -2.62855542280997 2.1649487284926]  x5=1.56768746601819e-07  V1=ones(3,3)  V2=ones(3,3)  I1=ones(3,3)  I2=ones(3,3)  nHarmo=1  Measurements=None
      settings: SourceProductName=Simscape Electrical
  54 : powerlib/Measurements/Three-Phase V-I Measurement  VoltageMeasurement=phase-to-ground  SetLabelV=on  LabelV=V54  Vpu=off  VpuLL=off  CurrentMeasurement=no  SetLabelI=on  LabelI=I65  Ipu=off  Pbase=100e6  Vbase=24900  OutputType=Complex  PhasorSimulation=on  PSBequivalent=0
      settings: SourceProductName=Simscape Electrical
  54-55 1 : powerlib/Elements/Distributed Parameters Line  Phases=3  Frequency=60  Resistance=R_1  Inductance=L_1  Capacitance=C_1  Length=275*ft2km  x1=[386.001754491217 4028.98439798237 4029.95524089406;376.991118430775 376.991118430775 376.991118430775;1.79155856549331 -2.42316850160712 2.27103908467448]  x2=[386.440764885173 4028.53772891639 4029.81234786367;376.991118430775 376.991118430775 376.991118430775;1.79326903972678 -2.42322750176539 2.27098478692169]  x3=[7.93929276524156 8.65048105864516 5.50622759360341;376.991118430775 376.991118430775 376.991118430775;1.60035805964398 -1.1090721234397 2.47020584722905]  x4=[6.94538155352765 29.1094520143959 18.3913370423307;376.991118430775 376.991118430775 376.991118430775;-1.5691311679597 -2.71480468606144 2.21166417977308]  x5=3.44891242524002e-07  V1=ones(3,3)  V2=ones(3,3)  I1=ones(3,3)  I2=ones(3,3)  nHarmo=1  Measurements=None
      settings: SourceProductName=Simscape Electrical
  54-57 3 : powerlib/Elements/Distributed Parameters Line  Phases=3  Frequency=60  Resistance=R_3  Inductance=L_3  Capacitance=C_3  Length=350*ft2km  x1=[403.236065920644 3995.89089045909 4062.15066688126;376.991118430775 376.991118430775 376.991118430775;-0.597676330497547 0.189941252554269 1.75270954459934]  x2=[402.855150485836 3983.13801060954 4051.99385201392;376.991118430775 376.991118430775 376.991118430775;-0.604886484113246 0.185448907660187 1.74907324629388]  x3=[21.0918543404844 423.104194025681 411.246164424247;376.991118430775 376.991118430775 376.991118430775;2.7976589330896 3.11697350568076 -1.49302458147796]  x4=[22.1180636575126 446.121991904526 441.386285691169;376.991118430775 376.991118430775 376.991118430775;-0.356129361493 -0.0135136669057854 1.65557268156073]  x5=4.38952490485094e-07  V1=ones(3,3)  V2=ones(3,3)  I1=ones(3,3)  I2=ones(3,3)  nHarmo=1  Measurements=None
      settings: SourceProductName=Simscape Electrical
  55 : powerlib/Measurements/Three-Phase V-I Measurement  VoltageMeasurement=phase-to-ground  SetLabelV=on  LabelV=V55  Vpu=off  VpuLL=off  CurrentMeasurement=no  SetLabelI=on  LabelI=I65  Ipu=off  Pbase=100e6  Vbase=24900  OutputType=Complex  PhasorSimulation=on  PSBequivalent=0
      settings: SourceProductName=Simscape Electrical
  55 Y Z : powerlib/Elements/Series RLC Load  LConnTagsString=a  RConnTagsString=__new0  NominalVoltage=1.0*2401.78  NominalFrequency=60  ActivePower=20e3*a  InductivePower=10e3*a  CapacitivePower=0  Setx0=off  InitialVoltage=0  SetiL0=off  InitialCurrent=0  Measurements=None  LoadType=constant Z
      settings: SourceProductName=Simscape Electrical
  55-56 1 : powerlib/Elements/Distributed Parameters Line  Phases=3  Frequency=60  Resistance=R_1  Inductance=L_1  Capacitance=C_1  Length=275*ft2km  x1=[386.440764885173 4028.53772891639 4029.81234786367;376.991118430775 376.991118430775 376.991118430775;1.79326903972678 -2.42322750176539 2.27098478692169]  x2=[387.229135797271 4028.32318588089 4029.68253428006;376.991118430775 376.991118430775 376.991118430775;1.79317524420031 -2.42329547628532 2.27100472135284]  x3=[7.58685152597791 4.92966062499062 12.99022658638;376.991118430775 376.991118430775 376.991118430775;0.621213423061808 -2.07516949449163 2.56781981615285]  x4=[7.25272392024528 25.4957137204124 11.9536672271463;376.991118430775 376.991118430775 376.991118430775;-2.64994302138095 -2.48932664585174 1.94742284241789]  x5=3.44891242524002e-07  V1=ones(3,3)  V2=ones(3,3)  I1=ones(3,3)  I2=ones(3,3)  nHarmo=1  Measurements=None
      settings: SourceProductName=Simscape Electrical
  56 : powerlib/Measurements/Three-Phase V-I Measurement  VoltageMeasurement=phase-to-ground  SetLabelV=on  LabelV=V56  Vpu=off  VpuLL=off  CurrentMeasurement=no  SetLabelI=on  LabelI=I65  Ipu=off  Pbase=100e6  Vbase=24900  OutputType=Complex  PhasorSimulation=on  PSBequivalent=0
      settings: SourceProductName=Simscape Electrical
  56 Y PQ : powerlib/Elements/Series RLC Load  LConnTagsString=a  RConnTagsString=__new0  NominalVoltage=1.0*2401.78  NominalFrequency=60  ActivePower=20e3*a  InductivePower=10e3*a  CapacitivePower=0  Setx0=off  InitialVoltage=0  SetiL0=off  InitialCurrent=0  Measurements=None  LoadType=constant PQ
      settings: SourceProductName=Simscape Electrical
  57 : powerlib/Measurements/Three-Phase V-I Measurement  VoltageMeasurement=phase-to-ground  SetLabelV=on  LabelV=V57  Vpu=off  VpuLL=off  CurrentMeasurement=no  SetLabelI=on  LabelI=I65  Ipu=off  Pbase=100e6  Vbase=24900  OutputType=Complex  PhasorSimulation=on  PSBequivalent=0
      settings: SourceProductName=Simscape Electrical
  57-58 10 : powerlib/Elements/Distributed Parameters Line  Phases=1  Frequency=60  Resistance=R_10(2,2)  Inductance=L_10(2,2)  Capacitance=C_10(2,2)  Length=250*ft2km  x1=[3332.65167546037;376.991118430775;-2.12346234184091]  x2=[3334.84331905035;376.991118430775;-2.12323827340863]  x3=[31.4123377270754;376.991118430775;-2.50011760545947]  x4=[20.5556871728064;376.991118430775;0.42119900823692]  x5=3.09938851618982e-07  V1=[2.049e+04;377;-2.115]  V2=[2.048e+04;377;-2.115]  I1=[33.62;377;-2.106]  I2=[35.2;377;-2.126]  nHarmo=1  Measurements=None
      settings: SourceProductName=Simscape Electrical
  57-60 3 : powerlib/Elements/Distributed Parameters Line  Phases=3  Frequency=60  Resistance=R_3  Inductance=L_3  Capacitance=C_3  Length=750*ft2km  x1=[402.855150485836 3983.13801060954 4051.99385201392;376.991118430775 376.991118430775 376.991118430775;-0.605075605473618 0.185292678993478 1.74891633512626]  x2=[405.241601073424 3956.13968740074 4031.72181002115;376.991118430775 376.991118430775 376.991118430775;-0.628148783828739 0.175994401394114 1.74102358362162]  x3=[32.6736209816878 410.216328849047 404.742315987075;376.991118430775 376.991118430775 376.991118430775;-3.11666579169372 3.09625697741235 -1.46083721631608]  x4=[33.5303525804294 433.05327479393 434.856467615936;376.991118430775 376.991118430775 376.991118430775;0.00596664524669986 -0.033235419901659 1.68519830568225]  x5=9.40612479610915e-07  V1=ones(3,3)  V2=ones(3,3)  I1=ones(3,3)  I2=ones(3,3)  nHarmo=1  Measurements=None
      settings: SourceProductName=Simscape Electrical
  58 : Subsystem
  58 Y I : powerlib/Elements/Series RLC Load  LConnTagsString=a  RConnTagsString=__new0  NominalVoltage=1.0*2401.78  NominalFrequency=60  ActivePower=20e3*a  InductivePower=10e3*a  CapacitivePower=0  Setx0=off  InitialVoltage=0  SetiL0=off  InitialCurrent=0  Measurements=None  LoadType=constant I
      settings: SourceProductName=Simscape Electrical
  58-59 10 : powerlib/Elements/Distributed Parameters Line  Phases=1  Frequency=60  Resistance=R_10(2,2)  Inductance=L_10(2,2)  Capacitance=C_10(2,2)  Length=10*ft2km  x1=[3332.60784409527;376.991118430775;-2.12335465559548]  x2=[3332.65167546037;376.991118430775;-2.12335017141436]  x3=[18.5785991357498;376.991118430775;-2.43955705072268]  x4=[7.94298526706756;376.991118430775;0.203811140638322]  x5=1.23975540647593e-08  V1=[2.049e+04;377;-2.115]  V2=[2.048e+04;377;-2.115]  I1=[33.62;377;-2.106]  I2=[35.2;377;-2.126]  nHarmo=1  Measurements=None
      settings: SourceProductName=Simscape Electrical
  59 : Subsystem
  59 Y PQ : powerlib/Elements/Series RLC Load  LConnTagsString=a  RConnTagsString=__new0  NominalVoltage=1.0*2401.78  NominalFrequency=60  ActivePower=20e3*a  InductivePower=10e3*a  CapacitivePower=0  Setx0=off  InitialVoltage=0  SetiL0=off  InitialCurrent=0  Measurements=None  LoadType=constant PQ
      settings: SourceProductName=Simscape Electrical
  59-94 : powerlib/Elements/Breaker  InitialState=0  SwitchingTimes="[1/60  5/60]"  External=off  BreakerResistance=0.01  SnubberResistance=1e6  SnubberCapacitance=inf  Measurements=None  MoreParameters=on  NoBreakLoop=off
      settings: SourceProductName=Simscape Electrical
  6 : Subsystem
  6 Y Z : powerlib/Elements/Series RLC Load  LConnTagsString=a  RConnTagsString=__new0  NominalVoltage=1.0*2401.78  NominalFrequency=60  ActivePower=40e3*a  InductivePower=20e3*a  CapacitivePower=0  Setx0=off  InitialVoltage=0  SetiL0=off  InitialCurrent=0  Measurements=None  LoadType=constant Z
      settings: SourceProductName=Simscape Electrical
  60 : powerlib/Measurements/Three-Phase V-I Measurement  VoltageMeasurement=phase-to-ground  SetLabelV=on  LabelV=V60  Vpu=off  VpuLL=off  CurrentMeasurement=no  SetLabelI=on  LabelI=I65  Ipu=off  Pbase=100e6  Vbase=24900  OutputType=Complex  PhasorSimulation=on  PSBequivalent=0
      settings: SourceProductName=Simscape Electrical
  60 Y PQ : powerlib/Elements/Series RLC Load  LConnTagsString=a  RConnTagsString=__new0  NominalVoltage=1.0*2401.78  NominalFrequency=60  ActivePower=20e3*a  InductivePower=10e3*a  CapacitivePower=0  Setx0=off  InitialVoltage=0  SetiL0=off  InitialCurrent=0  Measurements=None  LoadType=constant PQ
      settings: SourceProductName=Simscape Electrical
  60-1 : powerlib/Elements/Three-Phase Breaker  InitialState=closed  SwitchA=off  SwitchB=off  SwitchC=off  SwitchTimes="[1/60  5/60]"  External=off  BreakerResistance=0.01  SnubberResistance=1e6  SnubberCapacitance=inf  Measurements=None
      settings: SourceProductName=Simscape Electrical
  60-61 5 : powerlib/Elements/Distributed Parameters Line  Phases=3  Frequency=60  Resistance=R_5  Inductance=L_5  Capacitance=C_5  Length=550*ft2km  x1=[425.021901856439 3960.1369134924 4027.451392622;376.991118430775 376.991118430775 376.991118430775;2.61589227324382 0.269041261237203 1.83072227377314]  x2=[425.02146203275 3960.12674811166 4027.43929114404;376.991118430775 376.991118430775 376.991118430775;2.61589175401531 0.269040498467641 1.83072107988859]  x3=[0.556883232647686 14.6674303875884 11.7548020201363;376.991118430775 376.991118430775 376.991118430775;2.61850820100321 0.276616031872598 1.84041654252952]  x4=[0.560340986680023 14.8963279914312 11.9874139403465;376.991118430775 376.991118430775 376.991118430775;2.61303272398052 0.261368028612807 1.82100220760128]  x5=6.89782485048005e-07  V1=ones(3,3)  V2=ones(3,3)  I1=ones(3,3)  I2=ones(3,3)  nHarmo=1  Measurements=None
      settings: SourceProductName=Simscape Electrical
  60-62 12 : powerlib/Elements/Distributed Parameters Line  Phases=3  Frequency=60  Resistance=R_12  Inductance=L_12  Capacitance=C_12  Length=250*ft2km  x1=[123.581170502755 3980.68496340499 4009.41821082808;376.991118430775 376.991118430775 376.991118430775;-2.21275168337849 -0.57568127416098 -2.12845061955714]  x2=[123.207658831799 3974.71086464651 4004.88928615006;376.991118430775 376.991118430775 376.991118430775;-2.18824375096832 -0.57539161971298 -2.12855748306163]  x3=[22.9638893400141 80.7551731061618 43.3750715892438;376.991118430775 376.991118430775 376.991118430775;-1.0017997222418 1.54474859998764 0.338997219954678]  x4=[22.3711817792024 148.179824227353 136.771657397609;376.991118430775 376.991118430775 376.991118430775;2.21505515408212 -1.05899106303756 -2.32786699585039]  x5=1.15320558205325e-06  V1=ones(3,3)  V2=ones(3,3)  I1=ones(3,3)  I2=ones(3,3)  nHarmo=1  Measurements=None
      settings: SourceProductName=Simscape Electrical
  61 : powerlib/Measurements/Three-Phase V-I Measurement  VoltageMeasurement=phase-to-ground  SetLabelV=on  LabelV=V61  Vpu=off  VpuLL=off  CurrentMeasurement=no  SetLabelI=on  LabelI=I65  Ipu=off  Pbase=100e6  Vbase=24900  OutputType=Complex  PhasorSimulation=on  PSBequivalent=0
      settings: SourceProductName=Simscape Electrical
  61-610 : powerlib/Elements/Three-Phase Breaker  InitialState=closed  SwitchA=off  SwitchB=off  SwitchC=off  SwitchTimes="[1/60  5/60]"  External=off  BreakerResistance=0.01  SnubberResistance=1e6  SnubberCapacitance=inf  Measurements=None
      settings: SourceProductName=Simscape Electrical
  610 : powerlib/Measurements/Three-Phase V-I Measurement  VoltageMeasurement=phase-to-phase  SetLabelV=on  LabelV=V610  Vpu=off  VpuLL=off  CurrentMeasurement=no  SetLabelI=on  LabelI=I65  Ipu=off  Pbase=100e6  Vbase=24900  OutputType=Complex  PhasorSimulation=on  PSBequivalent=0
      settings: SourceProductName=Simscape Electrical
  62 : powerlib/Measurements/Three-Phase V-I Measurement  VoltageMeasurement=phase-to-ground  SetLabelV=on  LabelV=V62  Vpu=off  VpuLL=off  CurrentMeasurement=no  SetLabelI=on  LabelI=I65  Ipu=off  Pbase=100e6  Vbase=24900  OutputType=Complex  PhasorSimulation=on  PSBequivalent=0
      settings: SourceProductName=Simscape Electrical
  62 Y Z : powerlib/Elements/Series RLC Load  LConnTagsString=a  RConnTagsString=__new0  NominalVoltage=1.0*2401.78  NominalFrequency=60  ActivePower=40e3*a  InductivePower=20e3*a  CapacitivePower=0  Setx0=off  InitialVoltage=0  SetiL0=off  InitialCurrent=0  Measurements=None  LoadType=constant Z
      settings: SourceProductName=Simscape Electrical
  62-63 12 : powerlib/Elements/Distributed Parameters Line  Phases=3  Frequency=60  Resistance=R_12  Inductance=L_12  Capacitance=C_12  Length=175*ft2km  x1=[123.207658831799 3974.71086464651 4004.88928615006;376.991118430775 376.991118430775 376.991118430775;-2.18811332648967 -0.575306322345818 -2.12848112238545]  x2=[122.353612241193 3971.13374190371 4001.92830889063;376.991118430775 376.991118430775 376.991118430775;-2.18067156433342 -0.575184960123199 -2.12847714840006]  x3=[13.0537054107778 62.9807031371612 41.3561713196982;376.991118430775 376.991118430775 376.991118430775;-0.385636022992356 1.53219579281222 0.0963225487322859]  x4=[13.5734487202308 132.673771355638 129.485720710807;376.991118430775 376.991118430775 376.991118430775;2.88527889248651 -0.995552414256808 -2.38482980316733]  x5=8.07243907437275e-07  V1=ones(3,3)  V2=ones(3,3)  I1=ones(3,3)  I2=ones(3,3)  nHarmo=1  Measurements=None
      settings: SourceProductName=Simscape Electrical
  63 : powerlib/Measurements/Three-Phase V-I Measurement  VoltageMeasurement=phase-to-ground  SetLabelV=on  LabelV=V63  Vpu=off  VpuLL=off  CurrentMeasurement=no  SetLabelI=on  LabelI=I65  Ipu=off  Pbase=100e6  Vbase=24900  OutputType=Complex  PhasorSimulation=on  PSBequivalent=0
      settings: SourceProductName=Simscape Electrical
  63 Y PQ : powerlib/Elements/Series RLC Load  LConnTagsString=a  RConnTagsString=__new0  NominalVoltage=1.0*2401.78  NominalFrequency=60  ActivePower=40e3*a  InductivePower=20e3*a  CapacitivePower=0  Setx0=off  InitialVoltage=0  SetiL0=off  InitialCurrent=0  Measurements=None  LoadType=constant PQ
      settings: SourceProductName=Simscape Electrical
  63-64 12 : powerlib/Elements/Distributed Parameters Line  Phases=3  Frequency=60  Resistance=R_12  Inductance=L_12  Capacitance=C_12  Length=350*ft2km  x1=[122.353612241193 3971.13374190371 4001.92830889063;376.991118430775 376.991118430775 376.991118430775;-2.18097588811694 -0.575383987313243 -2.12865532331115]  x2=[119.328332153665 3965.13814927424 3996.32670529746;376.991118430775 376.991118430775 376.991118430775;-2.14650756899455 -0.574966126989617 -2.1288150726838]  x3=[27.1870588601128 57.066722329943 33.4946225521098;376.991118430775 376.991118430775 376.991118430775;-0.454784230750886 1.25635050329927 0.275308031006797]  x4=[27.4872031777917 117.284023513042 126.766742732325;376.991118430775 376.991118430775 376.991118430775;2.75053896387212 -1.06477684933466 -2.30750976766074]  x5=1.61448781487455e-06  V1=ones(3,3)  V2=ones(3,3)  I1=ones(3,3)  I2=ones(3,3)  nHarmo=1  Measurements=None
      settings: SourceProductName=Simscape Electrical
  64 : powerlib/Measurements/Three-Phase V-I Measurement  VoltageMeasurement=phase-to-ground  SetLabelV=on  LabelV=V64  Vpu=off  VpuLL=off  CurrentMeasurement=no  SetLabelI=on  LabelI=I65  Ipu=off  Pbase=100e6  Vbase=24900  OutputType=Complex  PhasorSimulation=on  PSBequivalent=0
      settings: SourceProductName=Simscape Electrical
  64 Y I : powerlib/Elements/Series RLC Load  LConnTagsString=a  RConnTagsString=__new0  NominalVoltage=1.0*2401.78  NominalFrequency=60  ActivePower=75e3*a  InductivePower=35e3*a  CapacitivePower=0  Setx0=off  InitialVoltage=0  SetiL0=off  InitialCurrent=0  Measurements=None  LoadType=constant I
      settings: SourceProductName=Simscape Electrical
  64-65 12 : powerlib/Elements/Distributed Parameters Line  Phases=3  Frequency=60  Resistance=R_12  Inductance=L_12  Capacitance=C_12  Length=425*ft2km  x1=[119.328332153665 3965.13814927424 3996.32670529746;376.991118430775 376.991118430775 376.991118430775;-2.14663799347319 -0.575051424356779 -2.12889143335997]  x2=[122.219898560559 3957.85787693018 3992.88222631752;376.991118430775 376.991118430775 376.991118430775;-2.10274942944914 -0.574541911417062 -2.12911145140512]  x3=[27.110924591391 57.1148432980391 11.7125422877031;376.991118430775 376.991118430775 376.991118430775;-1.52997316329895 1.25726709666508 -1.56031167481753]  x4=[25.6672737313391 117.200436632677 90.1833250514947;376.991118430775 376.991118430775 376.991118430775;1.65018568785945 -1.06518782260671 -2.19923997432769]  x5=1.96044948949052e-06  V1=ones(3,3)  V2=ones(3,3)  I1=ones(3,3)  I2=ones(3,3)  nHarmo=1  Measurements=None
      settings: SourceProductName=Simscape Electrical
  65 : powerlib/Measurements/Three-Phase V-I Measurement  VoltageMeasurement=phase-to-ground  SetLabelV=on  LabelV=V65  Vpu=off  VpuLL=off  CurrentMeasurement=yes  SetLabelI=on  LabelI=I65  Ipu=off  Pbase=100e6  Vbase=24900  OutputType=Complex  PhasorSimulation=on  PSBequivalent=0
      settings: SourceProductName=Simscape Electrical
  65 D Z : powerlib/Elements/Three-Phase Series RLC Load  LConnTagsString=A|B|C  Configuration=Delta  NominalVoltage=120e3  Vabc=[ 1.0 1.0 1.0]*2401.78  Vabcp=[ 1.0 1.0 1.0]*4160  NominalFrequency=60  UnbalancedPower=on  ActivePower=1e+006  InductivePower=0  CapacitivePower=0  Pabc="[17 66  117]*1e3/2"  QLabc="[10 38  68]*1e3/2"  QCabc=[0 0 0]  Pabcp=[35 35 70]*1e3*a  QLabcp=[25 25 50]*1e3*a  QCabcp=[0 0 0]  Measurements=None  LoadType=constant Z
      settings: SourceProductName=Simscape Electrical
  65-66 12 : powerlib/Elements/Distributed Parameters Line  Phases=3  Frequency=60  Resistance=R_12  Inductance=L_12  Capacitance=C_12  Length=325*ft2km  x1=[122.219898560559 3957.85787693018 3992.88222631753;376.991118430775 376.991118430775 376.991118430775;-2.10257553014428 -0.574428181594179 -2.12900963717022]  x2=[124.647378766667 3955.76817934148 3992.197108394;376.991118430775 376.991118430775 376.991118430775;-2.07054916036458 -0.574160789360823 -2.12928394817654]  x3=[27.2866823588094 36.6723324994051 35.7792350398462;376.991118430775 376.991118430775 376.991118430775;-1.54197345345598 0.239185758804672 -2.44097308920692]  x4=[25.7593619161611 68.7350798338201 66.6497666090781;376.991118430775 376.991118430775 376.991118430775;1.63594928862439 -0.972696647860256 -1.96394779790921]  x5=1.49916725666922e-06  V1=ones(3,3)  V2=ones(3,3)  I1=ones(3,3)  I2=ones(3,3)  nHarmo=1  Measurements=None
      settings: SourceProductName=Simscape Electrical
  66 : powerlib/Measurements/Three-Phase V-I Measurement  VoltageMeasurement=phase-to-ground  SetLabelV=on  LabelV=V66  Vpu=off  VpuLL=off  CurrentMeasurement=no  SetLabelI=on  LabelI=I65  Ipu=off  Pbase=100e6  Vbase=24900  OutputType=Complex  PhasorSimulation=on  PSBequivalent=0
      settings: SourceProductName=Simscape Electrical
  66 Y PQ : powerlib/Elements/Series RLC Load  LConnTagsString=a  RConnTagsString=__new0  NominalVoltage=1.0*2401.78  NominalFrequency=60  ActivePower=75e3*a  InductivePower=35e3*a  CapacitivePower=0  Setx0=off  InitialVoltage=0  SetiL0=off  InitialCurrent=0  Measurements=None  LoadType=constant PQ
      settings: SourceProductName=Simscape Electrical
  67 : powerlib/Measurements/Three-Phase V-I Measurement  VoltageMeasurement=phase-to-ground  SetLabelV=on  LabelV=V67  Vpu=off  VpuLL=off  CurrentMeasurement=no  SetLabelI=on  LabelI=I65  Ipu=off  Pbase=100e6  Vbase=24900  OutputType=Complex  PhasorSimulation=on  PSBequivalent=0
      settings: SourceProductName=Simscape Electrical
  67-68 9 : powerlib/Elements/Distributed Parameters Line  Phases=1  Frequency=60  Resistance=R_9(1,1)  Inductance=L_9(1,1)  Capacitance=C_9(1,1)  Length=200*ft2km  x1=[3194.90175039152;376.991118430775;-0.0591024421824385]  x2=[3189.87753877816;376.991118430775;-0.0596371896883663]  x3=[68.828789472223;376.991118430775;2.57940899709371]  x4=[79.2743337842407;376.991118430775;-0.49105664307475]  x5=2.47951081295186e-07  V1=[2.049e+04;377;-2.115]  V2=[2.048e+04;377;-2.115]  I1=[33.62;377;-2.106]  I2=[35.2;377;-2.126]  nHarmo=1  Measurements=None
      settings: SourceProductName=Simscape Electrical
  67-72 3 : powerlib/Elements/Distributed Parameters Line  Phases=3  Frequency=60  Resistance=R_3  Inductance=L_3  Capacitance=C_3  Length=275*ft2km  x1=[404.042933790345 3944.41227534201 4023.02675377783;376.991118430775 376.991118430775 376.991118430775;-0.642020648939171 0.172419543752611 1.73822778785991]  x2=[400.600700603361 3944.5332740135 4022.44591252667;376.991118430775 376.991118430775 376.991118430775;-0.639901768769328 0.170213794962756 1.73693728463462]  x3=[33.201190116779 208.27953696604 144.48935148725;376.991118430775 376.991118430775 376.991118430775;1.05275121660199 -2.52146498640297 -0.971371066881658]  x4=[33.3474531470996 229.450891545813 172.214245373941;376.991118430775 376.991118430775 376.991118430775;-2.05736147126228 0.576137245132817 2.09703364851184]  x5=3.44891242524002e-07  V1=ones(3,3)  V2=ones(3,3)  I1=ones(3,3)  I2=ones(3,3)  nHarmo=1  Measurements=None
      settings: SourceProductName=Simscape Electrical
  67-97 3 : powerlib/Elements/Distributed Parameters Line  Phases=3  Frequency=60  Resistance=R_3  Inductance=L_3  Capacitance=C_3  Length=250*ft2km  x1=[404.042933790345 3944.41227534201 4023.02675377783;376.991118430775 376.991118430775 376.991118430775;-0.642008828854148 0.17242930804428 1.73823759480789]  x2=[403.937531783188 3940.87502820857 4020.59041973766;376.991118430775 376.991118430775 376.991118430775;-0.64637919930311 0.171799804501433 1.73774876252717]  x3=[17.7505705845711 109.770972630403 90.6012866019646;376.991118430775 376.991118430775 376.991118430775;2.82869844225964 2.71149594543893 -1.85382250297182]  x4=[18.75796133131 129.595489918419 118.357986589119;376.991118430775 376.991118430775 376.991118430775;-0.331313650677943 -0.328336402722533 1.39837636396406]  x5=3.13537493203638e-07  V1=ones(3,3)  V2=ones(3,3)  I1=ones(3,3)  I2=ones(3,3)  nHarmo=1  Measurements=None
      settings: SourceProductName=Simscape Electrical
  68 : Subsystem
  68 Y PQ : powerlib/Elements/Series RLC Load  LConnTagsString=a  RConnTagsString=__new0  NominalVoltage=1.0*2401.78  NominalFrequency=60  ActivePower=20e3*a  InductivePower=10e3*a  CapacitivePower=0  Setx0=off  InitialVoltage=0  SetiL0=off  InitialCurrent=0  Measurements=None  LoadType=constant PQ
      settings: SourceProductName=Simscape Electrical
  68-69 9 : powerlib/Elements/Distributed Parameters Line  Phases=1  Frequency=60  Resistance=R_9(1,1)  Inductance=L_9(1,1)  Capacitance=C_9(1,1)  Length=275*ft2km  x1=[3189.87753877816;376.991118430775;-0.0596722429466614]  x2=[3184.12416874561;376.991118430775;-0.0602864561753862]  x3=[56.4816431768367;376.991118430775;2.57097961380172]  x4=[66.9085519781111;376.991118430775;-0.485262276989868]  x5=3.4093273678088e-07  V1=[2.049e+04;377;-2.115]  V2=[2.048e+04;377;-2.115]  I1=[33.62;377;-2.106]  I2=[35.2;377;-2.126]  nHarmo=1  Measurements=None
      settings: SourceProductName=Simscape Electrical
  69 : Subsystem
  69 Y PQ : powerlib/Elements/Series RLC Load  LConnTagsString=a  RConnTagsString=__new0  NominalVoltage=1.0*2401.78  NominalFrequency=60  ActivePower=40e3*a  InductivePower=20e3*a  CapacitivePower=0  Setx0=off  InitialVoltage=0  SetiL0=off  InitialCurrent=0  Measurements=None  LoadType=constant PQ
      settings: SourceProductName=Simscape Electrical
  69-70 9 : powerlib/Elements/Distributed Parameters Line  Phases=1  Frequency=60  Resistance=R_9(1,1)  Inductance=L_9(1,1)  Capacitance=C_9(1,1)  Length=325*ft2km  x1=[3184.12416874561;376.991118430775;-0.0603098250142496]  x2=[3180.04777789614;376.991118430775;-0.0607460874824776]  x3=[31.8528108943604;376.991118430775;2.53502881171918]  x4=[42.2479969042989;376.991118430775;-0.462842425976751]  x5=4.02920507104677e-07  V1=[2.049e+04;377;-2.115]  V2=[2.048e+04;377;-2.115]  I1=[33.62;377;-2.106]  I2=[35.2;377;-2.126]  nHarmo=1  Measurements=None
      settings: SourceProductName=Simscape Electrical
  7 : powerlib/Measurements/Three-Phase V-I Measurement  VoltageMeasurement=phase-to-ground  SetLabelV=on  LabelV=V7  Vpu=off  VpuLL=off  CurrentMeasurement=no  SetLabelI=on  LabelI=I800  Ipu=off  Pbase=100e6  Vbase=24900  OutputType=Complex  PhasorSimulation=on  PSBequivalent=0
      settings: SourceProductName=Simscape Electrical
  7 Y PQ : powerlib/Elements/Series RLC Load  LConnTagsString=a  RConnTagsString=__new0  NominalVoltage=1.0*2401.78  NominalFrequency=60  ActivePower=20e3*a  InductivePower=10e3*a  CapacitivePower=0  Setx0=off  InitialVoltage=0  SetiL0=off  InitialCurrent=0  Measurements=None  LoadType=constant PQ
      settings: SourceProductName=Simscape Electrical
  7-8 1 : powerlib/Elements/Distributed Parameters Line  Phases=3  Frequency=60  Resistance=R_1  Inductance=L_1  Capacitance=C_1  Length=200*ft2km  x1=[407.597893112689 4096.26742166794 4094.04240143975;376.991118430775 376.991118430775 376.991118430775;1.73959889707447 -2.4101052365278 2.29352703279485]  x2=[400.834100723123 4080.92323601732 4079.80081798922;376.991118430775 376.991118430775 376.991118430775;1.75442925341688 -2.41269626418302 2.28867448964288]  x3=[116.770064349706 763.055539340483 832.458346681532;376.991118430775 376.991118430775 376.991118430775;2.96980490027152 0.25900976806613 -1.06443871712511]  x4=[116.412103486301 790.375010743523 856.017211287719;376.991118430775 376.991118430775 376.991118430775;-0.163206941656182 -2.86505248348278 2.08312874062608]  x5=2.50829994562911e-07  V1=ones(3,3)  V2=ones(3,3)  I1=ones(3,3)  I2=ones(3,3)  nHarmo=1  Measurements=None
      settings: SourceProductName=Simscape Electrical
  70 : Subsystem
  70 Y PQ : powerlib/Elements/Series RLC Load  LConnTagsString=a  RConnTagsString=__new0  NominalVoltage=1.0*2401.78  NominalFrequency=60  ActivePower=20e3*a  InductivePower=10e3*a  CapacitivePower=0  Setx0=off  InitialVoltage=0  SetiL0=off  InitialCurrent=0  Measurements=None  LoadType=constant PQ
      settings: SourceProductName=Simscape Electrical
  70-71 1 : powerlib/Elements/Distributed Parameters Line  Phases=1  Frequency=60  Resistance=R_9(1,1)  Inductance=L_9(1,1)  Capacitance=C_9(1,1)  Length=275*ft2km  x1=[3180.04777789614;376.991118430775;-0.0607227186436142]  x2=[3177.74900349221;376.991118430775;-0.0609691811724815]  x3=[19.6000398433057;376.991118430775;2.48368189449247]  x4=[29.9522704111708;376.991118430775;-0.437624051783513]  x5=3.4093273678088e-07  V1=[2.049e+04;377;-2.115]  V2=[2.048e+04;377;-2.115]  I1=[33.62;377;-2.106]  I2=[35.2;377;-2.126]  nHarmo=1  Measurements=None
      settings: SourceProductName=Simscape Electrical
  71 : Subsystem
  71 Y PQ : powerlib/Elements/Series RLC Load  LConnTagsString=a  RConnTagsString=__new0  NominalVoltage=1.0*2401.78  NominalFrequency=60  ActivePower=40e3*a  InductivePower=20e3*a  CapacitivePower=0  Setx0=off  InitialVoltage=0  SetiL0=off  InitialCurrent=0  Measurements=None  LoadType=constant PQ
      settings: SourceProductName=Simscape Electrical
  72 : powerlib/Measurements/Three-Phase V-I Measurement  VoltageMeasurement=phase-to-ground  SetLabelV=on  LabelV=V72  Vpu=off  VpuLL=off  CurrentMeasurement=no  SetLabelI=on  LabelI=I65  Ipu=off  Pbase=100e6  Vbase=24900  OutputType=Complex  PhasorSimulation=on  PSBequivalent=0
      settings: SourceProductName=Simscape Electrical
  72-73 11 : powerlib/Elements/Distributed Parameters Line  Phases=1  Frequency=60  Resistance=R_11(3,3)  Inductance=L_11(3,3)  Capacitance=C_11(3,3)  Length=275*ft2km  x1=[3258.10363795756;376.991118430775;2.05311512253186]  x2=[3251.0575501703;376.991118430775;2.05237909489368]  x3=[70.2055023175657;376.991118430775;-1.59147202092582]  x4=[80.8551852446649;376.991118430775;1.62118711642622]  x5=3.4093273678088e-07  V1=[2.049e+04;377;-2.115]  V2=[2.048e+04;377;-2.115]  I1=[33.62;377;-2.106]  I2=[35.2;377;-2.126]  nHarmo=1  Measurements=None
      settings: SourceProductName=Simscape Electrical
  72-76 3 : powerlib/Elements/Distributed Parameters Line  Phases=3  Frequency=60  Resistance=R_3  Inductance=L_3  Capacitance=C_3  Length=200*ft2km  x1=[400.600700603361 3944.5332740135 4022.44591252667;376.991118430775 376.991118430775 376.991118430775;-0.639866308514258 0.170243087837764 1.73696670547855]  x2=[398.09840287341 3944.63329842317 4022.02766104051;376.991118430775 376.991118430775 376.991118430775;-0.638302284704393 0.168639000401818 1.73602792862476]  x3=[33.2031399702622 208.291123880924 144.499897752053;376.991118430775 376.991118430775 376.991118430775;1.05291640814581 -2.5213292660937 -0.971236394060366]  x4=[33.346406209969 229.444949557067 172.208867994072;376.991118430775 376.991118430775 376.991118430775;-2.05742095640991 0.576087753561206 2.0969829921379]  x5=2.50829994562911e-07  V1=ones(3,3)  V2=ones(3,3)  I1=ones(3,3)  I2=ones(3,3)  nHarmo=1  Measurements=None
      settings: SourceProductName=Simscape Electrical
  73 : Subsystem
  73 Y PQ : powerlib/Elements/Series RLC Load  LConnTagsString=a  RConnTagsString=__new0  NominalVoltage=1.0*2401.78  NominalFrequency=60  ActivePower=40e3*a  InductivePower=20e3*a  CapacitivePower=0  Setx0=off  InitialVoltage=0  SetiL0=off  InitialCurrent=0  Measurements=None  LoadType=constant PQ
      settings: SourceProductName=Simscape Electrical
  73-74 11 : powerlib/Elements/Distributed Parameters Line  Phases=1  Frequency=60  Resistance=R_11(3,3)  Inductance=L_11(3,3)  Capacitance=C_11(3,3)  Length=350*ft2km  x1=[3251.0575501703;376.991118430775;2.05234404163539]  x2=[3245.0845982561;376.991118430775;2.05171801795446]  x3=[45.0408119239632;376.991118430775;-1.61289849404658]  x4=[55.6627439492243;376.991118430775;1.63568583867945]  x5=4.33914392266575e-07  V1=[2.049e+04;377;-2.115]  V2=[2.048e+04;377;-2.115]  I1=[33.62;377;-2.106]  I2=[35.2;377;-2.126]  nHarmo=1  Measurements=None
      settings: SourceProductName=Simscape Electrical
  74 : Subsystem
  74 Y Z : powerlib/Elements/Series RLC Load  LConnTagsString=a  RConnTagsString=__new0  NominalVoltage=1.0*2401.78  NominalFrequency=60  ActivePower=40e3*a  InductivePower=20e3*a  CapacitivePower=0  Setx0=off  InitialVoltage=0  SetiL0=off  InitialCurrent=0  Measurements=None  LoadType=constant Z
      settings: SourceProductName=Simscape Electrical
  74-75 11 : powerlib/Elements/Distributed Parameters Line  Phases=1  Frequency=60  Resistance=R_11(3,3)  Inductance=L_11(3,3)  Capacitance=C_11(3,3)  Length=400*ft2km  x1=[3245.0845982561;376.991118430775;2.05169464911559]  x2=[3241.67361645119;376.991118430775;2.05133627061289]  x3=[19.9923810407149;376.991118430775;-1.68726370245516]  x4=[30.5538405724387;376.991118430775;1.67468029872325]  x5=4.95902162590371e-07  V1=[2.049e+04;377;-2.115]  V2=[2.048e+04;377;-2.115]  I1=[33.62;377;-2.106]  I2=[35.2;377;-2.126]  nHarmo=1  Measurements=None
      settings: SourceProductName=Simscape Electrical
  75 : Subsystem
  75 Y PQ : powerlib/Elements/Series RLC Load  LConnTagsString=a  RConnTagsString=__new0  NominalVoltage=1.0*2401.78  NominalFrequency=60  ActivePower=40e3*a  InductivePower=20e3*a  CapacitivePower=0  Setx0=off  InitialVoltage=0  SetiL0=off  InitialCurrent=0  Measurements=None  LoadType=constant PQ
      settings: SourceProductName=Simscape Electrical
  76 : powerlib/Measurements/Three-Phase V-I Measurement  VoltageMeasurement=phase-to-ground  SetLabelV=on  LabelV=V76  Vpu=off  VpuLL=off  CurrentMeasurement=no  SetLabelI=on  LabelI=I65  Ipu=off  Pbase=100e6  Vbase=24900  OutputType=Complex  PhasorSimulation=on  PSBequivalent=0
      settings: SourceProductName=Simscape Electrical
  76 DI : powerlib/Elements/Three-Phase Series RLC Load  LConnTagsString=A|B|C  Configuration=Delta  NominalVoltage=120e3  Vabc=[ 1.0 1.0 1.0]*2401.78  Vabcp=[ 1.0 1.0 1.0]*4160  NominalFrequency=60  UnbalancedPower=on  ActivePower=1e+006  InductivePower=0  CapacitivePower=0  Pabc="[17 66  117]*1e3/2"  QLabc="[10 38  68]*1e3/2"  QCabc=[0 0 0]  Pabcp="[105 70  70]*1e3*a"  QLabcp=[80 50 50]*1e3*a  QCabcp=[0 0 0]  Measurements=None  LoadType=constant I
      settings: SourceProductName=Simscape Electrical
  76-77 6 : powerlib/Elements/Distributed Parameters Line  Phases=3  Frequency=60  Resistance=R_6  Inductance=L_6  Capacitance=C_6  Length=400*ft2km  x1=[483.988690884173 3990.77648421217 3975.34145763837;376.991118430775 376.991118430775 376.991118430775;-1.82695619134996 2.3432643301217 -2.35013528942489]  x2=[484.356746621959 3994.15678752493 3979.924416529;376.991118430775 376.991118430775 376.991118430775;-1.82798248029799 2.34203147002044 -2.35152623208516]  x3=[3.69477982215322 118.429305304448 119.383264626291;376.991118430775 376.991118430775 376.991118430775;2.48028171914293 0.41980282904827 1.98216785554002]  x4=[4.35580266769406 131.710325461747 129.904641925406;376.991118430775 376.991118430775 376.991118430775;-0.933257866730442 -2.93583994724963 -1.32789138931495]  x5=5.01659989125821e-07  V1=ones(3,3)  V2=ones(3,3)  I1=ones(3,3)  I2=ones(3,3)  nHarmo=1  Measurements=None
      settings: SourceProductName=Simscape Electrical
  76-86 3 : powerlib/Elements/Distributed Parameters Line  Phases=3  Frequency=60  Resistance=R_3  Inductance=L_3  Capacitance=C_3  Length=700*ft2km  x1=[398.09840287341 3944.63329842317 4022.02766104051;376.991118430775 376.991118430775 376.991118430775;-0.638538686404858 0.168443714568431 1.73583178966523]  x2=[389.725132711134 3943.58441849279 4019.51592014074;376.991118430775 376.991118430775 376.991118430775;-0.630433829528464 0.166392572269579 1.73514537080832]  x3=[33.0210937710145 69.4981406708534 30.0121853253871;376.991118430775 376.991118430775 376.991118430775;0.937719599258916 -2.64462662560379 -1.75650119245775]  x4=[33.038997578178 91.8044954272716 59.1088576445216;376.991118430775 376.991118430775 376.991118430775;-2.17252883643412 0.414885968266965 1.56022928272809]  x5=8.77904980970188e-07  V1=ones(3,3)  V2=ones(3,3)  I1=ones(3,3)  I2=ones(3,3)  nHarmo=1  Measurements=None
      settings: SourceProductName=Simscape Electrical
  77 : powerlib/Measurements/Three-Phase V-I Measurement  VoltageMeasurement=phase-to-ground  SetLabelV=on  LabelV=V77  Vpu=off  VpuLL=off  CurrentMeasurement=no  SetLabelI=on  LabelI=I65  Ipu=off  Pbase=100e6  Vbase=24900  OutputType=Complex  PhasorSimulation=on  PSBequivalent=0
      settings: SourceProductName=Simscape Electrical
  77 Y PQ : powerlib/Elements/Series RLC Load  LConnTagsString=a  RConnTagsString=__new0  NominalVoltage=1.0*2401.78  NominalFrequency=60  ActivePower=40e3*a  InductivePower=20e3*a  CapacitivePower=0  Setx0=off  InitialVoltage=0  SetiL0=off  InitialCurrent=0  Measurements=None  LoadType=constant PQ
      settings: SourceProductName=Simscape Electrical
  77-78 6 : powerlib/Elements/Distributed Parameters Line  Phases=3  Frequency=60  Resistance=R_6  Inductance=L_6  Capacitance=C_6  Length=100*ft2km  x1=[484.356746621959 3994.15678752493 3979.924416529;376.991118430775 376.991118430775 376.991118430775;-1.82784063927771 2.34214915339616 -2.35140906058513]  x2=[484.987080258944 3995.03451093566 3981.24184436217;376.991118430775 376.991118430775 376.991118430775;-1.82760799908545 2.34183407455485 -2.35170139514203]  x3=[16.8676574633804 121.984540302433 118.490273253989;376.991118430775 376.991118430775 376.991118430775;-2.80798043160608 0.423544761658973 2.14360454666725]  x4=[16.1928217862579 135.086026946539 125.654454643412;376.991118430775 376.991118430775 376.991118430775;0.268209415361401 -2.92712785530007 -1.18137801634767]  x5=1.25414997281455e-07  V1=ones(3,3)  V2=ones(3,3)  I1=ones(3,3)  I2=ones(3,3)  nHarmo=1  Measurements=None
      settings: SourceProductName=Simscape Electrical
  78 : powerlib/Measurements/Three-Phase V-I Measurement  VoltageMeasurement=phase-to-ground  SetLabelV=on  LabelV=V78  Vpu=off  VpuLL=off  CurrentMeasurement=no  SetLabelI=on  LabelI=I65  Ipu=off  Pbase=100e6  Vbase=24900  OutputType=Complex  PhasorSimulation=on  PSBequivalent=0
      settings: SourceProductName=Simscape Electrical
  78-79 6 : powerlib/Elements/Distributed Parameters Line  Phases=3  Frequency=60  Resistance=R_6  Inductance=L_6  Capacitance=C_6  Length=225*ft2km  x1=[484.987080258944 3995.03451093566 3981.24184436217;376.991118430775 376.991118430775 376.991118430775;-1.82766709951056 2.34178503981497 -2.35175021660038]  x2=[485.989586995047 3994.94729777046 3980.76352813861;376.991118430775 376.991118430775 376.991118430775;-1.82924007398599 2.34169243600798 -2.35173106806596]  x3=[14.2943196045772 4.02812185228191 16.4792831459753;376.991118430775 376.991118430775 376.991118430775;2.65746805339419 1.1151540031286 -1.2875636861156]  x4=[14.6337525502929 28.7166609253403 21.1434583511411;376.991118430775 376.991118430775 376.991118430775;-0.569212300209714 2.47412243379055 -3.10162097657115]  x5=2.82183743883275e-07  V1=ones(3,3)  V2=ones(3,3)  I1=ones(3,3)  I2=ones(3,3)  nHarmo=1  Measurements=None
      settings: SourceProductName=Simscape Electrical
  78-80 6 : powerlib/Elements/Distributed Parameters Line  Phases=3  Frequency=60  Resistance=R_6  Inductance=L_6  Capacitance=C_6  Length=475*ft2km  x1=[484.987080258944 3995.03451093566 3981.24184436217;376.991118430775 376.991118430775 376.991118430775;-1.8277853003608 2.34168697033521 -2.35184785951707]  x2=[485.870825776972 3999.39205115083 3988.5141540553;376.991118430775 376.991118430775 376.991118430775;-1.82336213735052 2.34038760039324 -2.35327379212343]  x3=[13.2491146073044 114.377064166983 131.927468752609;376.991118430775 376.991118430775 376.991118430775;-1.83419347990391 0.523724714279579 2.19471114858556]  x4=[11.9731475108009 125.050637374374 137.749209437903;376.991118430775 376.991118430775 376.991118430775;1.30649230078302 -2.85140026096335 -1.11589845017909]  x5=5.95721237086913e-07  V1=ones(3,3)  V2=ones(3,3)  I1=ones(3,3)  I2=ones(3,3)  nHarmo=1  Measurements=None
      settings: SourceProductName=Simscape Electrical
  79 : powerlib/Measurements/Three-Phase V-I Measurement  VoltageMeasurement=phase-to-ground  SetLabelV=on  LabelV=V79  Vpu=off  VpuLL=off  CurrentMeasurement=no  SetLabelI=on  LabelI=I65  Ipu=off  Pbase=100e6  Vbase=24900  OutputType=Complex  PhasorSimulation=on  PSBequivalent=0
      settings: SourceProductName=Simscape Electrical
  79 Y Z : powerlib/Elements/Series RLC Load  LConnTagsString=a  RConnTagsString=__new0  NominalVoltage=1.0*2401.78  NominalFrequency=60  ActivePower=40e3*a  InductivePower=20e3*a  CapacitivePower=0  Setx0=off  InitialVoltage=0  SetiL0=off  InitialCurrent=0  Measurements=None  LoadType=constant Z
      settings: SourceProductName=Simscape Electrical
  8 : powerlib/Measurements/Three-Phase V-I Measurement  VoltageMeasurement=phase-to-ground  SetLabelV=on  LabelV=V8  Vpu=off  VpuLL=off  CurrentMeasurement=no  SetLabelI=on  LabelI=I800  Ipu=off  Pbase=100e6  Vbase=24900  OutputType=Complex  PhasorSimulation=on  PSBequivalent=0
      settings: SourceProductName=Simscape Electrical
  8-12 10 : powerlib/Elements/Distributed Parameters Line  Phases=1  Frequency=60  Resistance=R_10(2,2)  Inductance=L_10(2,2)  Capacitance=C_10(2,2)  Length=225*ft2km  x1=[3368.25023180577;376.991118430775;-2.10735674164618]  x2=[3367.25377487692;376.991118430775;-2.10745761241105]  x3=[8.02405309660832;376.991118430775;0.219566144430136]  x4=[18.7706674789597;376.991118430775;-2.42366253700172]  x5=2.78944966457084e-07  V1=[2.049e+04;377;-2.115]  V2=[2.048e+04;377;-2.115]  I1=[33.62;377;-2.106]  I2=[35.2;377;-2.126]  nHarmo=1  Measurements=None
      settings: SourceProductName=Simscape Electrical
  8-13 1 : powerlib/Elements/Distributed Parameters Line  Phases=3  Frequency=60  Resistance=R_1  Inductance=L_1  Capacitance=C_1  Length=300*ft2km  x1=[400.834100723123 4080.92323601732 4079.80081798922;376.991118430775 376.991118430775 376.991118430775;1.75438197307678 -2.41273549197492 2.28863543247621]  x2=[392.068269812946 4059.48221006893 4058.82663428491;376.991118430775 376.991118430775 376.991118430775;1.76792684169291 -2.416630690917 2.28168027726913]  x3=[88.4939013404706 726.704938821586 800.344635146277;376.991118430775 376.991118430775 376.991118430775;-3.12522239704037 0.288365981060279 -1.08570733413203]  x4=[88.3196106898309 754.326355246284 823.72373440798;376.991118430775 376.991118430775 376.991118430775;0.0279922258462332 -2.8361232049823 2.06250250491875]  x5=3.76244991844366e-07  V1=ones(3,3)  V2=ones(3,3)  I1=ones(3,3)  I2=ones(3,3)  nHarmo=1  Measurements=None
      settings: SourceProductName=Simscape Electrical
  8-9 9 : powerlib/Elements/Distributed Parameters Line  Phases=1  Frequency=60  Resistance=R_9(1,1)  Inductance=L_9(1,1)  Capacitance=C_9(1,1)  Length=225*ft2km  x1=[3298.1557552422;376.991118430775;-0.0220456900127539]  x2=[3293.2882092088;376.991118430775;-0.022548187945782]  x3=[58.4053107130974;376.991118430775;2.60866715383102]  x4=[69.1880918794864;376.991118430775;-0.447568591484376]  x5=2.78944966457084e-07  V1=[2.049e+04;377;-2.115]  V2=[2.048e+04;377;-2.115]  I1=[33.62;377;-2.106]  I2=[35.2;377;-2.126]  nHarmo=1  Measurements=None
      settings: SourceProductName=Simscape Electrical
  80 : powerlib/Measurements/Three-Phase V-I Measurement  VoltageMeasurement=phase-to-ground  SetLabelV=on  LabelV=V80  Vpu=off  VpuLL=off  CurrentMeasurement=no  SetLabelI=on  LabelI=I65  Ipu=off  Pbase=100e6  Vbase=24900  OutputType=Complex  PhasorSimulation=on  PSBequivalent=0
      settings: SourceProductName=Simscape Electrical
  80 Y PQ : powerlib/Elements/Series RLC Load  LConnTagsString=a  RConnTagsString=__new0  NominalVoltage=1.0*2401.78  NominalFrequency=60  ActivePower=40e3*a  InductivePower=20e3*a  CapacitivePower=0  Setx0=off  InitialVoltage=0  SetiL0=off  InitialCurrent=0  Measurements=None  LoadType=constant PQ
      settings: SourceProductName=Simscape Electrical
  80-81 6 : powerlib/Elements/Distributed Parameters Line  Phases=3  Frequency=60  Resistance=R_6  Inductance=L_6  Capacitance=C_6  Length=475*ft2km  x1=[485.870825776972 3999.39205115083 3988.5141540553;376.991118430775 376.991118430775 376.991118430775;-1.82336213735052 2.34038760039324 -2.35327379212343]  x2=[489.338635109724 4003.90732188973 3996.60448003067;376.991118430775 376.991118430775 376.991118430775;-1.81670424162533 2.33905697383015 -2.35443392292025]  x3=[26.382576804258 117.961245739378 134.9571140146;376.991118430775 376.991118430775 376.991118430775;-2.24670315537536 0.524319610032088 2.33716860820933]  x4=[25.2212747625287 128.504514034136 137.486291954679;376.991118430775 376.991118430775 376.991118430775;0.873861355730671 -2.84478404681325 -0.976417630343468]  x5=5.95721237086913e-07  V1=ones(3,3)  V2=ones(3,3)  I1=ones(3,3)  I2=ones(3,3)  nHarmo=1  Measurements=None
      settings: SourceProductName=Simscape Electrical
  81 : powerlib/Measurements/Three-Phase V-I Measurement  VoltageMeasurement=phase-to-ground  SetLabelV=on  LabelV=V81  Vpu=off  VpuLL=off  CurrentMeasurement=no  SetLabelI=on  LabelI=I65  Ipu=off  Pbase=100e6  Vbase=24900  OutputType=Complex  PhasorSimulation=on  PSBequivalent=0
      settings: SourceProductName=Simscape Electrical
  81-82 6 : powerlib/Elements/Distributed Parameters Line  Phases=3  Frequency=60  Resistance=R_6  Inductance=L_6  Capacitance=C_6  Length=250*ft2km  x1=[489.338635109724 4003.90732188973 3996.60448003067;376.991118430775 376.991118430775 376.991118430775;-1.81659786086012 2.33914523636193 -2.35434604429523]  x2=[490.906568464602 4007.16725471396 4000.71332346551;376.991118430775 376.991118430775 376.991118430775;-1.81736795745771 2.33851623306297 -2.35486065333579]  x3=[16.7488989856703 135.811986633292 127.043535106146;376.991118430775 376.991118430775 376.991118430775;3.07870435069041 0.723335357529815 2.39811978415198]  x4=[16.5624995154123 140.36256640172 128.272787484462;376.991118430775 376.991118430775 376.991118430775;-0.139449292188089 -2.63272875496716 -0.928137846646562]  x5=3.13537493203638e-07  V1=ones(3,3)  V2=ones(3,3)  I1=ones(3,3)  I2=ones(3,3)  nHarmo=1  Measurements=None
      settings: SourceProductName=Simscape Electrical
  81-84 11 : powerlib/Elements/Distributed Parameters Line  Phases=1  Frequency=60  Resistance=R_11(3,3)  Inductance=L_11(3,3)  Capacitance=C_11(3,3)  Length=675*ft2km  x1=[3269.85018081927;376.991118430775;2.04532502854731]  x2=[3261.17003331985;376.991118430775;2.04442077071894]  x3=[32.6436987843015;376.991118430775;-1.6433212406403]  x4=[43.3082697402307;376.991118430775;1.64224891099538]  x5=8.36834899371251e-07  V1=[2.049e+04;377;-2.115]  V2=[2.048e+04;377;-2.115]  I1=[33.62;377;-2.106]  I2=[35.2;377;-2.126]  nHarmo=1  Measurements=None
      settings: SourceProductName=Simscape Electrical
  82 : powerlib/Measurements/Three-Phase V-I Measurement  VoltageMeasurement=phase-to-ground  SetLabelV=on  LabelV=V82  Vpu=off  VpuLL=off  CurrentMeasurement=no  SetLabelI=on  LabelI=I65  Ipu=off  Pbase=100e6  Vbase=24900  OutputType=Complex  PhasorSimulation=on  PSBequivalent=0
      settings: SourceProductName=Simscape Electrical
  82 Y PQ : powerlib/Elements/Series RLC Load  LConnTagsString=a  RConnTagsString=__new0  NominalVoltage=1.0*2401.78  NominalFrequency=60  ActivePower=40e3*a  InductivePower=20e3*a  CapacitivePower=0  Setx0=off  InitialVoltage=0  SetiL0=off  InitialCurrent=0  Measurements=None  LoadType=constant PQ
      settings: SourceProductName=Simscape Electrical
  82-83 6 : powerlib/Elements/Distributed Parameters Line  Phases=3  Frequency=60  Resistance=R_6  Inductance=L_6  Capacitance=C_6  Length=250*ft2km  x1=[490.906568464602 4007.16725471396 4000.71332346551;376.991118430775 376.991118430775 376.991118430775;-1.81736795745771 2.33851623306297 -2.35486065333579]  x2=[491.36726260486 4010.52579252785 4005.35748815836;376.991118430775 376.991118430775 376.991118430775;-1.81636731650123 2.33799130509027 -2.35539536532794]  x3=[7.55695132566529 132.090453270731 141.709892588453;376.991118430775 376.991118430775 376.991118430775;-2.15748931144422 0.825353349170301 2.42057638324183]  x4=[6.35468384130483 133.737403222877 142.17966135545;376.991118430775 376.991118430775 376.991118430775;0.916189543182736 -2.54154708160173 -0.887424017788122]  x5=3.13537493203638e-07  V1=ones(3,3)  V2=ones(3,3)  I1=ones(3,3)  I2=ones(3,3)  nHarmo=1  Measurements=None
      settings: SourceProductName=Simscape Electrical
  83 : powerlib/Measurements/Three-Phase V-I Measurement  VoltageMeasurement=phase-to-ground  SetLabelV=on  LabelV=V83  Vpu=off  VpuLL=off  CurrentMeasurement=no  SetLabelI=on  LabelI=I65  Ipu=off  Pbase=100e6  Vbase=24900  OutputType=Complex  PhasorSimulation=on  PSBequivalent=0
      settings: SourceProductName=Simscape Electrical
  83 Y CAP : powerlib/Elements/Three-Phase Series RLC Load  LConnTagsString=A|B|C  Configuration=Y (grounded)  NominalVoltage=120e3  Vabc=[ 1.0 1.0 1.0]*2401.78  Vabcp=[1e3 1e3 1e3]  NominalFrequency=60  UnbalancedPower=on  ActivePower=1e+006  InductivePower=0  CapacitivePower=0  Pabc=[0 0 0 ]*1e3  QLabc=[0 0 0 ]*1e3  QCabc=[200 200 200]*1e3*a  Pabcp=[10e3 9e3 11e3]  QLabcp=[100 90 110]  QCabcp=[100 90 110]  Measurements=None  LoadType=constant Z
      settings: SourceProductName=Simscape Electrical
  83 Y PQ : powerlib/Elements/Series RLC Load  LConnTagsString=a  RConnTagsString=__new0  NominalVoltage=1.0*2401.78  NominalFrequency=60  ActivePower=20e3*a  InductivePower=10e3*a  CapacitivePower=0  Setx0=off  InitialVoltage=0  SetiL0=off  InitialCurrent=0  Measurements=None  LoadType=constant PQ
      settings: SourceProductName=Simscape Electrical
  84 : Subsystem
  84 Y PQ : powerlib/Elements/Series RLC Load  LConnTagsString=a  RConnTagsString=__new0  NominalVoltage=1.0*2401.78  NominalFrequency=60  ActivePower=20e3*a  InductivePower=10e3*a  CapacitivePower=0  Setx0=off  InitialVoltage=0  SetiL0=off  InitialCurrent=0  Measurements=None  LoadType=constant PQ
      settings: SourceProductName=Simscape Electrical
  84-85 11 : powerlib/Elements/Distributed Parameters Line  Phases=1  Frequency=60  Resistance=R_11(3,3)  Inductance=L_11(3,3)  Capacitance=C_11(3,3)  Length=475*ft2km  x1=[3261.17003331985;376.991118430775;2.04451424607439]  x2=[3257.10018272013;376.991118430775;2.04408875162538]  x3=[20.086351520727;376.991118430775;-1.69455060799637]  x4=[30.6986623558489;376.991118430775;1.66743216207573]  x5=5.88883818076066e-07  V1=[2.049e+04;377;-2.115]  V2=[2.048e+04;377;-2.115]  I1=[33.62;377;-2.106]  I2=[35.2;377;-2.126]  nHarmo=1  Measurements=None
      settings: SourceProductName=Simscape Electrical
  85 : Subsystem
  85 Y PQ : powerlib/Elements/Series RLC Load  LConnTagsString=a  RConnTagsString=__new0  NominalVoltage=1.0*2401.78  NominalFrequency=60  ActivePower=40e3*a  InductivePower=20e3*a  CapacitivePower=0  Setx0=off  InitialVoltage=0  SetiL0=off  InitialCurrent=0  Measurements=None  LoadType=constant PQ
      settings: SourceProductName=Simscape Electrical
